simulink model "K_Sim_SG_Load"  (R2020b)
settings: Solver=FixedStepAuto  StartTime=0  StopTime=10  FixedStep=Ts  RelTol=1e-3
undefined symbols (not defined in the file or in its folder): DeviceDiscreDamping, DevicePara, DevicePowerFlow, DeviceType, Fbase, OtherInputs, Sbase, Ts, Vbase, Wbase, x_e, Ybase, Zbase
libraries: powerlib x222, SimplexPS x84
(part 1 of 2)
settings Model: Creator=admin_user  LastModifiedBy=admin_user

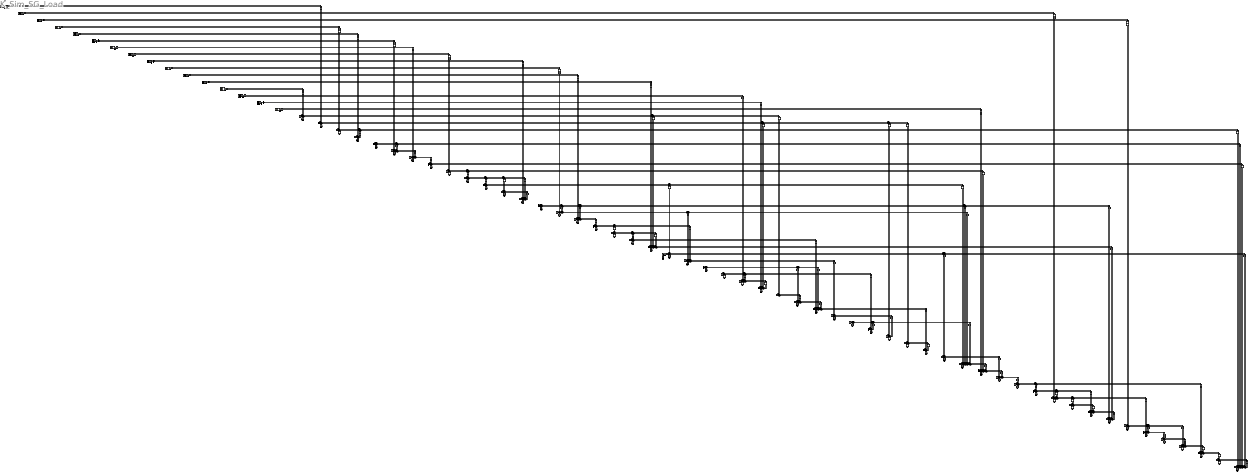
== system K_Sim_SG_Load ==
  note: Short-Circuit Fault
  B-GND{17,20,24,27..28,31,33,35,37,40,44,47,49..50,55,58,60,63,66,68,70,73,75,78,81,83,85,87,89,91,94..96,98..99,101,103,105,107,110,113,116,118,120..121,124,126,128,130,132,134} (51 alike) : powerlib/Elements/Ground  LConnTagsString=a
  Branch1-18 : powerlib/Elements/Three-Phase Series RLC Branch  LConnTagsString=A|B|C  RConnTagsString=A|B|C  BranchType=RL  Resistance=(1e-07)*Zbase  Inductance=(0.003)*Zbase/Wbase  Capacitance=1e-6  Measurements=None
  Branch10-31 : powerlib/Elements/Three-Phase Series RLC Branch  LConnTagsString=A|B|C  RConnTagsString=A|B|C  BranchType=RL  Resistance=(1e-07)*Zbase  Inductance=(0.026)*Zbase/Wbase  Capacitance=1e-6  Measurements=None
  Branch11-32 : powerlib/Elements/Three-Phase Series RLC Branch  LConnTagsString=A|B|C  RConnTagsString=A|B|C  BranchType=RL  Resistance=(1e-07)*Zbase  Inductance=(0.013)*Zbase/Wbase  Capacitance=1e-6  Measurements=None
  Branch12-36 : powerlib/Elements/Three-Phase Series RLC Branch  LConnTagsString=A|B|C  RConnTagsString=A|B|C  BranchType=RL  Resistance=(1e-07)*Zbase  Inductance=(0.0075)*Zbase/Wbase  Capacitance=1e-6  Measurements=None
  Branch13-17 : powerlib/Elements/Three-Phase Series RLC Branch  LConnTagsString=A|B|C  RConnTagsString=A|B|C  BranchType=RL  Resistance=(1e-07)*Zbase  Inductance=(0.0033)*Zbase/Wbase  Capacitance=1e-6  Measurements=None
  Branch14-41 : powerlib/Elements/Three-Phase Series RLC Branch  LConnTagsString=A|B|C  RConnTagsString=A|B|C  BranchType=RL  Resistance=(1e-07)*Zbase  Inductance=(0.0015)*Zbase/Wbase  Capacitance=1e-6  Measurements=None
  Branch15-42 : powerlib/Elements/Three-Phase Series RLC Branch  LConnTagsString=A|B|C  RConnTagsString=A|B|C  BranchType=RL  Resistance=(1e-07)*Zbase  Inductance=(0.0015)*Zbase/Wbase  Capacitance=1e-6  Measurements=None
  Branch16-54 : powerlib/Elements/Three-Phase Series RLC Branch  LConnTagsString=A|B|C  RConnTagsString=A|B|C  BranchType=RL  Resistance=(1e-07)*Zbase  Inductance=(0.0181)*Zbase/Wbase  Capacitance=1e-6  Measurements=None
  Branch17-17 : powerlib/Elements/Three-Phase Parallel RLC Branch  LConnTagsString=A|B|C  RConnTagsString=A|B|C  BranchType=RLC  Resistance=(0.015039)*Zbase  Inductance=(0.30078)*Zbase/Wbase  Capacitance=(0.16)*Ybase/Wbase  Measurements=None
      settings: SourceProductBaseCode=PS
  Branch17-36 : powerlib/Elements/Three-Phase Series RLC Branch  LConnTagsString=A|B|C  RConnTagsString=A|B|C  BranchType=RL  Resistance=(0.0005)*Zbase  Inductance=(0.0045)*Zbase/Wbase  Capacitance=1e-6  Measurements=None
  Branch17-43 : powerlib/Elements/Three-Phase Series RLC Branch  LConnTagsString=A|B|C  RConnTagsString=A|B|C  BranchType=RL  Resistance=(0.0005)*Zbase  Inductance=(0.0276)*Zbase/Wbase  Capacitance=1e-6  Measurements=None
  Branch18-18 : powerlib/Elements/Three-Phase Parallel RLC Branch  LConnTagsString=A|B|C  RConnTagsString=A|B|C  BranchType=RLC  Resistance=(0.040675)*Zbase  Inductance=(0.8168)*Zbase/Wbase  Capacitance=(2.735)*Ybase/Wbase  Measurements=None
      settings: SourceProductBaseCode=PS
  Branch18-42 : powerlib/Elements/Three-Phase Series RLC Branch  LConnTagsString=A|B|C  RConnTagsString=A|B|C  BranchType=RL  Resistance=(0.004)*Zbase  Inductance=(0.06)*Zbase/Wbase  Capacitance=1e-6  Measurements=None
  Branch18-49 : powerlib/Elements/Three-Phase Series RLC Branch  LConnTagsString=A|B|C  RConnTagsString=A|B|C  BranchType=RL  Resistance=(0.0076)*Zbase  Inductance=(0.1141)*Zbase/Wbase  Capacitance=1e-6  Measurements=None
  Branch18-50 : powerlib/Elements/Three-Phase Series RLC Branch  LConnTagsString=A|B|C  RConnTagsString=A|B|C  BranchType=RL  Resistance=(0.0012)*Zbase  Inductance=(0.0288)*Zbase/Wbase  Capacitance=1e-6  Measurements=None
  Branch19-19 : powerlib/Elements/Three-Phase Parallel RLC Branch  LConnTagsString=A|B|C  RConnTagsString=A|B|C  BranchType=C  Resistance=(Inf)*Zbase  Inductance=1e-3  Capacitance=(0.152)*Ybase/Wbase  Measurements=None
      settings: SourceProductBaseCode=PS
  Branch19-20 : powerlib/Elements/Three-Phase Series RLC Branch  LConnTagsString=A|B|C  RConnTagsString=A|B|C  BranchType=RL  Resistance=(0.00078652)*Zbase  Inductance=(0.015506)*Zbase/Wbase  Capacitance=1e-6  Measurements=None
  Branch19-68 : powerlib/Elements/Three-Phase Series RLC Branch  LConnTagsString=A|B|C  RConnTagsString=A|B|C  BranchType=RL  Resistance=(0.0016)*Zbase  Inductance=(0.0195)*Zbase/Wbase  Capacitance=1e-6  Measurements=None
  Branch2-58 : powerlib/Elements/Three-Phase Series RLC Branch  LConnTagsString=A|B|C  RConnTagsString=A|B|C  BranchType=RL  Resistance=(1e-07)*Zbase  Inductance=(0.025)*Zbase/Wbase  Capacitance=1e-6  Measurements=None
  Branch20-20 : powerlib/Elements/Three-Phase Parallel RLC Branch  LConnTagsString=A|B|C  RConnTagsString=A|B|C  BranchType=RL  Resistance=(0.14141)*Zbase  Inductance=(0.93359)*Zbase/Wbase  Capacitance=(0)*Ybase/Wbase  Measurements=None
      settings: SourceProductBaseCode=PS
  Branch21-21 : powerlib/Elements/Three-Phase Parallel RLC Branch  LConnTagsString=A|B|C  RConnTagsString=A|B|C  BranchType=RLC  Resistance=(0.33652)*Zbase  Inductance=(0.8018)*Zbase/Wbase  Capacitance=(0.25565)*Ybase/Wbase  Measurements=None
      settings: SourceProductBaseCode=PS
  Branch21-22 : powerlib/Elements/Three-Phase Series RLC Branch  LConnTagsString=A|B|C  RConnTagsString=A|B|C  BranchType=RL  Resistance=(0.0008)*Zbase  Inductance=(0.014)*Zbase/Wbase  Capacitance=1e-6  Measurements=None
  Branch21-68 : powerlib/Elements/Three-Phase Series RLC Branch  LConnTagsString=A|B|C  RConnTagsString=A|B|C  BranchType=RL  Resistance=(0.0008)*Zbase  Inductance=(0.0135)*Zbase/Wbase  Capacitance=1e-6  Measurements=None
  Branch22-22 : powerlib/Elements/Three-Phase Parallel RLC Branch  LConnTagsString=A|B|C  RConnTagsString=A|B|C  BranchType=C  Resistance=(Inf)*Zbase  Inductance=1e-3  Capacitance=(0.22055)*Ybase/Wbase  Measurements=None
      settings: SourceProductBaseCode=PS
  Branch22-23 : powerlib/Elements/Three-Phase Series RLC Branch  LConnTagsString=A|B|C  RConnTagsString=A|B|C  BranchType=RL  Resistance=(0.0006)*Zbase  Inductance=(0.0096)*Zbase/Wbase  Capacitance=1e-6  Measurements=None
  Branch23-23 : powerlib/Elements/Three-Phase Parallel RLC Branch  LConnTagsString=A|B|C  RConnTagsString=A|B|C  BranchType=RLC  Resistance=(0.40009)*Zbase  Inductance=(1.1673)*Zbase/Wbase  Capacitance=(0.2728)*Ybase/Wbase  Measurements=None
      settings: SourceProductBaseCode=PS
  Branch23-24 : powerlib/Elements/Three-Phase Series RLC Branch  LConnTagsString=A|B|C  RConnTagsString=A|B|C  BranchType=RL  Resistance=(0.0022)*Zbase  Inductance=(0.035)*Zbase/Wbase  Capacitance=1e-6  Measurements=None
  Branch24-24 : powerlib/Elements/Three-Phase Parallel RLC Branch  LConnTagsString=A|B|C  RConnTagsString=A|B|C  BranchType=RC  Resistance=(0.29745)*Zbase  Inductance=1e-3  Capacitance=(1.2155)*Ybase/Wbase  Measurements=None
      settings: SourceProductBaseCode=PS
  Branch24-68 : powerlib/Elements/Three-Phase Series RLC Branch  LConnTagsString=A|B|C  RConnTagsString=A|B|C  BranchType=RL  Resistance=(0.0003)*Zbase  Inductance=(0.0059)*Zbase/Wbase  Capacitance=1e-6  Measurements=None
  Branch25-25 : powerlib/Elements/Three-Phase Parallel RLC Branch  LConnTagsString=A|B|C  RConnTagsString=A|B|C  BranchType=RLC  Resistance=(0.44474)*Zbase  Inductance=(2.1196)*Zbase/Wbase  Capacitance=(0.3385)*Ybase/Wbase  Measurements=None
      settings: SourceProductBaseCode=PS
  Branch25-26 : powerlib/Elements/Three-Phase Series RLC Branch  LConnTagsString=A|B|C  RConnTagsString=A|B|C  BranchType=RL  Resistance=(0.0032)*Zbase  Inductance=(0.0323)*Zbase/Wbase  Capacitance=1e-6  Measurements=None
  Branch25-54 : powerlib/Elements/Three-Phase Series RLC Branch  LConnTagsString=A|B|C  RConnTagsString=A|B|C  BranchType=RL  Resistance=(0.007)*Zbase  Inductance=(0.0086)*Zbase/Wbase  Capacitance=1e-6  Measurements=None
  Branch26-26 : powerlib/Elements/Three-Phase Parallel RLC Branch  LConnTagsString=A|B|C  RConnTagsString=A|B|C  BranchType=RLC  Resistance=(0.70064)*Zbase  Inductance=(5.7288)*Zbase/Wbase  Capacitance=(1.2899)*Ybase/Wbase  Measurements=None
      settings: SourceProductBaseCode=PS
  Branch26-27 : powerlib/Elements/Three-Phase Series RLC Branch  LConnTagsString=A|B|C  RConnTagsString=A|B|C  BranchType=RL  Resistance=(0.0014)*Zbase  Inductance=(0.0147)*Zbase/Wbase  Capacitance=1e-6  Measurements=None
  Branch26-28 : powerlib/Elements/Three-Phase Series RLC Branch  LConnTagsString=A|B|C  RConnTagsString=A|B|C  BranchType=RL  Resistance=(0.0043)*Zbase  Inductance=(0.0474)*Zbase/Wbase  Capacitance=1e-6  Measurements=None
  Branch26-29 : powerlib/Elements/Three-Phase Series RLC Branch  LConnTagsString=A|B|C  RConnTagsString=A|B|C  BranchType=RL  Resistance=(0.0057)*Zbase  Inductance=(0.0625)*Zbase/Wbase  Capacitance=1e-6  Measurements=None
  Branch27-27 : powerlib/Elements/Three-Phase Parallel RLC Branch  LConnTagsString=A|B|C  RConnTagsString=A|B|C  BranchType=RLC  Resistance=(0.33339)*Zbase  Inductance=(1.2327)*Zbase/Wbase  Capacitance=(0.4856)*Ybase/Wbase  Measurements=None
      settings: SourceProductBaseCode=PS
  Branch27-37 : powerlib/Elements/Three-Phase Series RLC Branch  LConnTagsString=A|B|C  RConnTagsString=A|B|C  BranchType=RL  Resistance=(0.0013)*Zbase  Inductance=(0.0173)*Zbase/Wbase  Capacitance=1e-6  Measurements=None
  Branch27-53 : powerlib/Elements/Three-Phase Series RLC Branch  LConnTagsString=A|B|C  RConnTagsString=A|B|C  BranchType=RL  Resistance=(0.032)*Zbase  Inductance=(0.32)*Zbase/Wbase  Capacitance=1e-6  Measurements=None
  Branch28-28 : powerlib/Elements/Three-Phase Parallel RLC Branch  LConnTagsString=A|B|C  RConnTagsString=A|B|C  BranchType=RLC  Resistance=(0.47552)*Zbase  Inductance=(3.4985)*Zbase/Wbase  Capacitance=(0.5146)*Ybase/Wbase  Measurements=None
      settings: SourceProductBaseCode=PS
  Branch28-29 : powerlib/Elements/Three-Phase Series RLC Branch  LConnTagsString=A|B|C  RConnTagsString=A|B|C  BranchType=RL  Resistance=(0.0014)*Zbase  Inductance=(0.0151)*Zbase/Wbase  Capacitance=1e-6  Measurements=None
  Branch29-29 : powerlib/Elements/Three-Phase Parallel RLC Branch  LConnTagsString=A|B|C  RConnTagsString=A|B|C  BranchType=RLC  Resistance=(0.34656)*Zbase  Inductance=(3.6453)*Zbase/Wbase  Capacitance=(0.639)*Ybase/Wbase  Measurements=None
      settings: SourceProductBaseCode=PS
  Branch3-62 : powerlib/Elements/Three-Phase Series RLC Branch  LConnTagsString=A|B|C  RConnTagsString=A|B|C  BranchType=RL  Resistance=(1e-07)*Zbase  Inductance=(0.02)*Zbase/Wbase  Capacitance=1e-6  Measurements=None
  Branch30-30 : powerlib/Elements/Three-Phase Parallel RLC Branch  LConnTagsString=A|B|C  RConnTagsString=A|B|C  BranchType=C  Resistance=(Inf)*Zbase  Inductance=1e-3  Capacitance=(0.9405)*Ybase/Wbase  Measurements=None
      settings: SourceProductBaseCode=PS
  Branch30-31 : powerlib/Elements/Three-Phase Series RLC Branch  LConnTagsString=A|B|C  RConnTagsString=A|B|C  BranchType=RL  Resistance=(0.0013)*Zbase  Inductance=(0.0187)*Zbase/Wbase  Capacitance=1e-6  Measurements=None
  Branch30-32 : powerlib/Elements/Three-Phase Series RLC Branch  LConnTagsString=A|B|C  RConnTagsString=A|B|C  BranchType=RL  Resistance=(0.0024)*Zbase  Inductance=(0.0288)*Zbase/Wbase  Capacitance=1e-6  Measurements=None
  Branch30-53 : powerlib/Elements/Three-Phase Series RLC Branch  LConnTagsString=A|B|C  RConnTagsString=A|B|C  BranchType=RL  Resistance=(0.0008)*Zbase  Inductance=(0.0074)*Zbase/Wbase  Capacitance=1e-6  Measurements=None
  Branch30-61 : powerlib/Elements/Three-Phase Series RLC Branch  LConnTagsString=A|B|C  RConnTagsString=A|B|C  BranchType=RL  Resistance=(0.00095)*Zbase  Inductance=(0.00915)*Zbase/Wbase  Capacitance=1e-6  Measurements=None
  Branch31-31 : powerlib/Elements/Three-Phase Parallel RLC Branch  LConnTagsString=A|B|C  RConnTagsString=A|B|C  BranchType=C  Resistance=(Inf)*Zbase  Inductance=1e-3  Capacitance=(0.415)*Ybase/Wbase  Measurements=None
      settings: SourceProductBaseCode=PS
  Branch31-38 : powerlib/Elements/Three-Phase Series RLC Branch  LConnTagsString=A|B|C  RConnTagsString=A|B|C  BranchType=RL  Resistance=(0.0011)*Zbase  Inductance=(0.0147)*Zbase/Wbase  Capacitance=1e-6  Measurements=None
  Branch31-53 : powerlib/Elements/Three-Phase Series RLC Branch  LConnTagsString=A|B|C  RConnTagsString=A|B|C  BranchType=RL  Resistance=(0.0016)*Zbase  Inductance=(0.0163)*Zbase/Wbase  Capacitance=1e-6  Measurements=None
  Branch32-32 : powerlib/Elements/Three-Phase Parallel RLC Branch  LConnTagsString=A|B|C  RConnTagsString=A|B|C  BranchType=C  Resistance=(Inf)*Zbase  Inductance=1e-3  Capacitance=(0.328)*Ybase/Wbase  Measurements=None
      settings: SourceProductBaseCode=PS
  Branch32-33 : powerlib/Elements/Three-Phase Series RLC Branch  LConnTagsString=A|B|C  RConnTagsString=A|B|C  BranchType=RL  Resistance=(0.0008)*Zbase  Inductance=(0.0099)*Zbase/Wbase  Capacitance=1e-6  Measurements=None
  Branch33-33 : powerlib/Elements/Three-Phase Parallel RLC Branch  LConnTagsString=A|B|C  RConnTagsString=A|B|C  BranchType=RC  Resistance=(0.8467)*Zbase  Inductance=1e-3  Capacitance=(0.5315)*Ybase/Wbase  Measurements=None
      settings: SourceProductBaseCode=PS
  Branch33-34 : powerlib/Elements/Three-Phase Series RLC Branch  LConnTagsString=A|B|C  RConnTagsString=A|B|C  BranchType=RL  Resistance=(0.0011)*Zbase  Inductance=(0.0157)*Zbase/Wbase  Capacitance=1e-6  Measurements=None
  Branch33-38 : powerlib/Elements/Three-Phase Series RLC Branch  LConnTagsString=A|B|C  RConnTagsString=A|B|C  BranchType=RL  Resistance=(0.0036)*Zbase  Inductance=(0.0444)*Zbase/Wbase  Capacitance=1e-6  Measurements=None
  Branch34-34 : powerlib/Elements/Three-Phase Parallel RLC Branch  LConnTagsString=A|B|C  RConnTagsString=A|B|C  BranchType=C  Resistance=(Inf)*Zbase  Inductance=1e-3  Capacitance=(0.826)*Ybase/Wbase  Measurements=None
      settings: SourceProductBaseCode=PS
  Branch34-35 : powerlib/Elements/Three-Phase Series RLC Branch  LConnTagsString=A|B|C  RConnTagsString=A|B|C  BranchType=RL  Resistance=(0.0001)*Zbase  Inductance=(0.0074)*Zbase/Wbase  Capacitance=1e-6  Measurements=None
  Branch34-36 : powerlib/Elements/Three-Phase Series RLC Branch  LConnTagsString=A|B|C  RConnTagsString=A|B|C  BranchType=RL  Resistance=(0.0033)*Zbase  Inductance=(0.0111)*Zbase/Wbase  Capacitance=1e-6  Measurements=None
  Branch35-35 : powerlib/Elements/Three-Phase Parallel RLC Branch  LConnTagsString=A|B|C  RConnTagsString=A|B|C  BranchType=C  Resistance=(Inf)*Zbase  Inductance=1e-3  Capacitance=(0.695)*Ybase/Wbase  Measurements=None
      settings: SourceProductBaseCode=PS
  Branch35-45 : powerlib/Elements/Three-Phase Series RLC Branch  LConnTagsString=A|B|C  RConnTagsString=A|B|C  BranchType=RL  Resistance=(0.0007)*Zbase  Inductance=(0.0175)*Zbase/Wbase  Capacitance=1e-6  Measurements=None
  Branch36-36 : powerlib/Elements/Three-Phase Parallel RLC Branch  LConnTagsString=A|B|C  RConnTagsString=A|B|C  BranchType=RC  Resistance=(0.90473)*Zbase  Inductance=1e-3  Capacitance=(1.4359)*Ybase/Wbase  Measurements=None
      settings: SourceProductBaseCode=PS
  Branch36-61 : powerlib/Elements/Three-Phase Series RLC Branch  LConnTagsString=A|B|C  RConnTagsString=A|B|C  BranchType=RL  Resistance=(0.0011)*Zbase  Inductance=(0.0098)*Zbase/Wbase  Capacitance=1e-6  Measurements=None
  Branch37-37 : powerlib/Elements/Three-Phase Parallel RLC Branch  LConnTagsString=A|B|C  RConnTagsString=A|B|C  BranchType=C  Resistance=(Inf)*Zbase  Inductance=1e-3  Capacitance=(0.29385)*Ybase/Wbase  Measurements=None
      settings: SourceProductBaseCode=PS
  Branch37-52 : powerlib/Elements/Three-Phase Series RLC Branch  LConnTagsString=A|B|C  RConnTagsString=A|B|C  BranchType=RL  Resistance=(0.0007)*Zbase  Inductance=(0.0082)*Zbase/Wbase  Capacitance=1e-6  Measurements=None
  Branch37-68 : powerlib/Elements/Three-Phase Series RLC Branch  LConnTagsString=A|B|C  RConnTagsString=A|B|C  BranchType=RL  Resistance=(0.0007)*Zbase  Inductance=(0.0089)*Zbase/Wbase  Capacitance=1e-6  Measurements=None
  Branch38-38 : powerlib/Elements/Three-Phase Parallel RLC Branch  LConnTagsString=A|B|C  RConnTagsString=A|B|C  BranchType=C  Resistance=(Inf)*Zbase  Inductance=1e-3  Capacitance=(0.685)*Ybase/Wbase  Measurements=None
      settings: SourceProductBaseCode=PS
  Branch38-46 : powerlib/Elements/Three-Phase Series RLC Branch  LConnTagsString=A|B|C  RConnTagsString=A|B|C  BranchType=RL  Resistance=(0.0022)*Zbase  Inductance=(0.0284)*Zbase/Wbase  Capacitance=1e-6  Measurements=None
  Branch39-39 : powerlib/Elements/Three-Phase Parallel RLC Branch  LConnTagsString=A|B|C  RConnTagsString=A|B|C  BranchType=RL  Resistance=(0.36822)*Zbase  Inductance=(7.8028)*Zbase/Wbase  Capacitance=(0)*Ybase/Wbase  Measurements=None
      settings: SourceProductBaseCode=PS
  Branch39-44 : powerlib/Elements/Three-Phase Series RLC Branch  LConnTagsString=A|B|C  RConnTagsString=A|B|C  BranchType=RL  Resistance=(1e-07)*Zbase  Inductance=(0.0411)*Zbase/Wbase  Capacitance=1e-6  Measurements=None
  Branch39-45 : powerlib/Elements/Three-Phase Series RLC Branch  LConnTagsString=A|B|C  RConnTagsString=A|B|C  BranchType=RL  Resistance=(1e-07)*Zbase  Inductance=(0.0839)*Zbase/Wbase  Capacitance=1e-6  Measurements=None
  Branch4-19 : powerlib/Elements/Three-Phase Series RLC Branch  LConnTagsString=A|B|C  RConnTagsString=A|B|C  BranchType=RL  Resistance=(0.0007)*Zbase  Inductance=(0.0142)*Zbase/Wbase  Capacitance=1e-6  Measurements=None
  Branch40-40 : powerlib/Elements/Three-Phase Parallel RLC Branch  LConnTagsString=A|B|C  RConnTagsString=A|B|C  BranchType=RLC  Resistance=(1.6614)*Zbase  Inductance=(4.6341)*Zbase/Wbase  Capacitance=(2.215)*Ybase/Wbase  Measurements=None
      settings: SourceProductBaseCode=PS
  Branch40-41 : powerlib/Elements/Three-Phase Series RLC Branch  LConnTagsString=A|B|C  RConnTagsString=A|B|C  BranchType=RL  Resistance=(0.006)*Zbase  Inductance=(0.084)*Zbase/Wbase  Capacitance=1e-6  Measurements=None
  Branch40-48 : powerlib/Elements/Three-Phase Series RLC Branch  LConnTagsString=A|B|C  RConnTagsString=A|B|C  BranchType=RL  Resistance=(0.002)*Zbase  Inductance=(0.022)*Zbase/Wbase  Capacitance=1e-6  Measurements=None
  Branch41-41 : powerlib/Elements/Three-Phase Parallel RLC Branch  LConnTagsString=A|B|C  RConnTagsString=A|B|C  BranchType=RLC  Resistance=(0.099929)*Zbase  Inductance=(0.39972)*Zbase/Wbase  Capacitance=(2.7)*Ybase/Wbase  Measurements=None
      settings: SourceProductBaseCode=PS
  Branch41-42 : powerlib/Elements/Three-Phase Series RLC Branch  LConnTagsString=A|B|C  RConnTagsString=A|B|C  BranchType=RL  Resistance=(0.004)*Zbase  Inductance=(0.06)*Zbase/Wbase  Capacitance=1e-6  Measurements=None
  Branch42-42 : powerlib/Elements/Three-Phase Parallel RLC Branch  LConnTagsString=A|B|C  RConnTagsString=A|B|C  BranchType=RLC  Resistance=(0.086776)*Zbase  Inductance=(0.39917)*Zbase/Wbase  Capacitance=(2.25)*Ybase/Wbase  Measurements=None
      settings: SourceProductBaseCode=PS
  Branch43-44 : powerlib/Elements/Three-Phase Series RLC Branch  LConnTagsString=A|B|C  RConnTagsString=A|B|C  BranchType=RL  Resistance=(0.0001)*Zbase  Inductance=(0.0011)*Zbase/Wbase  Capacitance=1e-6  Measurements=None
  Branch44-44 : powerlib/Elements/Three-Phase Parallel RLC Branch  LConnTagsString=A|B|C  RConnTagsString=A|B|C  BranchType=RL  Resistance=(0.35712)*Zbase  Inductance=(19.7413)*Zbase/Wbase  Capacitance=(0)*Ybase/Wbase  Measurements=None
      settings: SourceProductBaseCode=PS
  Branch44-45 : powerlib/Elements/Three-Phase Series RLC Branch  LConnTagsString=A|B|C  RConnTagsString=A|B|C  BranchType=RL  Resistance=(0.0025)*Zbase  Inductance=(0.073)*Zbase/Wbase  Capacitance=1e-6  Measurements=None
  Branch45-45 : powerlib/Elements/Three-Phase Parallel RLC Branch  LConnTagsString=A|B|C  RConnTagsString=A|B|C  BranchType=RLC  Resistance=(0.52711)*Zbase  Inductance=(5.2209)*Zbase/Wbase  Capacitance=(1.055)*Ybase/Wbase  Measurements=None
      settings: SourceProductBaseCode=PS
  Branch45-51 : powerlib/Elements/Three-Phase Series RLC Branch  LConnTagsString=A|B|C  RConnTagsString=A|B|C  BranchType=RL  Resistance=(0.0004)*Zbase  Inductance=(0.0105)*Zbase/Wbase  Capacitance=1e-6  Measurements=None
  Branch46-46 : powerlib/Elements/Three-Phase Parallel RLC Branch  LConnTagsString=A|B|C  RConnTagsString=A|B|C  BranchType=RLC  Resistance=(0.65078)*Zbase  Inductance=(3.4411)*Zbase/Wbase  Capacitance=(0.35)*Ybase/Wbase  Measurements=None
      settings: SourceProductBaseCode=PS
  Branch46-49 : powerlib/Elements/Three-Phase Series RLC Branch  LConnTagsString=A|B|C  RConnTagsString=A|B|C  BranchType=RL  Resistance=(0.0018)*Zbase  Inductance=(0.0274)*Zbase/Wbase  Capacitance=1e-6  Measurements=None
  Branch47-47 : powerlib/Elements/Three-Phase Parallel RLC Branch  LConnTagsString=A|B|C  RConnTagsString=A|B|C  BranchType=RLC  Resistance=(0.5106)*Zbase  Inductance=(3.1824)*Zbase/Wbase  Capacitance=(1.055)*Ybase/Wbase  Measurements=None
      settings: SourceProductBaseCode=PS
  Branch47-48 : powerlib/Elements/Three-Phase Series RLC Branch  LConnTagsString=A|B|C  RConnTagsString=A|B|C  BranchType=RL  Resistance=(0.00125)*Zbase  Inductance=(0.0134)*Zbase/Wbase  Capacitance=1e-6  Measurements=None
  Branch47-53 : powerlib/Elements/Three-Phase Series RLC Branch  LConnTagsString=A|B|C  RConnTagsString=A|B|C  BranchType=RL  Resistance=(0.0013)*Zbase  Inductance=(0.0188)*Zbase/Wbase  Capacitance=1e-6  Measurements=None
  Branch48-48 : powerlib/Elements/Three-Phase Parallel RLC Branch  LConnTagsString=A|B|C  RConnTagsString=A|B|C  BranchType=RLC  Resistance=(0.44304)*Zbase  Inductance=(48.5738)*Zbase/Wbase  Capacitance=(1.04)*Ybase/Wbase  Measurements=None
      settings: SourceProductBaseCode=PS
  Branch49-49 : powerlib/Elements/Three-Phase Parallel RLC Branch  LConnTagsString=A|B|C  RConnTagsString=A|B|C  BranchType=RLC  Resistance=(0.60199)*Zbase  Inductance=(3.4044)*Zbase/Wbase  Capacitance=(0.715)*Ybase/Wbase  Measurements=None
      settings: SourceProductBaseCode=PS
  Branch5-20 : powerlib/Elements/Three-Phase Series RLC Branch  LConnTagsString=A|B|C  RConnTagsString=A|B|C  BranchType=RL  Resistance=(0.0009)*Zbase  Inductance=(0.018)*Zbase/Wbase  Capacitance=1e-6  Measurements=None
  Branch50-50 : powerlib/Elements/Three-Phase Parallel RLC Branch  LConnTagsString=A|B|C  RConnTagsString=A|B|C  BranchType=RC  Resistance=(1.1241)*Zbase  Inductance=1e-3  Capacitance=(3.1477)*Ybase/Wbase  Measurements=None
      settings: SourceProductBaseCode=PS
  Branch50-51 : powerlib/Elements/Three-Phase Series RLC Branch  LConnTagsString=A|B|C  RConnTagsString=A|B|C  BranchType=RL  Resistance=(0.0009)*Zbase  Inductance=(0.0221)*Zbase/Wbase  Capacitance=1e-6  Measurements=None
  Branch51-51 : powerlib/Elements/Three-Phase Parallel RLC Branch  LConnTagsString=A|B|C  RConnTagsString=A|B|C  BranchType=RC  Resistance=(0.33554)*Zbase  Inductance=1e-3  Capacitance=(2.2489)*Ybase/Wbase  Measurements=None
      settings: SourceProductBaseCode=PS
  Branch52-52 : powerlib/Elements/Three-Phase Parallel RLC Branch  LConnTagsString=A|B|C  RConnTagsString=A|B|C  BranchType=RLC  Resistance=(0.57667)*Zbase  Inductance=(3.0371)*Zbase/Wbase  Capacitance=(0.17285)*Ybase/Wbase  Measurements=None
      settings: SourceProductBaseCode=PS
  Branch52-55 : powerlib/Elements/Three-Phase Series RLC Branch  LConnTagsString=A|B|C  RConnTagsString=A|B|C  BranchType=RL  Resistance=(0.0011)*Zbase  Inductance=(0.0133)*Zbase/Wbase  Capacitance=1e-6  Measurements=None
  Branch53-53 : powerlib/Elements/Three-Phase Parallel RLC Branch  LConnTagsString=A|B|C  RConnTagsString=A|B|C  BranchType=RLC  Resistance=(0.38498)*Zbase  Inductance=(0.82056)*Zbase/Wbase  Capacitance=(1.5744)*Ybase/Wbase  Measurements=None
      settings: SourceProductBaseCode=PS
  Branch53-54 : powerlib/Elements/Three-Phase Series RLC Branch  LConnTagsString=A|B|C  RConnTagsString=A|B|C  BranchType=RL  Resistance=(0.0035)*Zbase  Inductance=(0.0411)*Zbase/Wbase  Capacitance=1e-6  Measurements=None
  Branch54-54 : powerlib/Elements/Three-Phase Parallel RLC Branch  LConnTagsString=A|B|C  RConnTagsString=A|B|C  BranchType=C  Resistance=(Inf)*Zbase  Inductance=1e-3  Capacitance=(0.55095)*Ybase/Wbase  Measurements=None
      settings: SourceProductBaseCode=PS
  Branch54-55 : powerlib/Elements/Three-Phase Series RLC Branch  LConnTagsString=A|B|C  RConnTagsString=A|B|C  BranchType=RL  Resistance=(0.0013)*Zbase  Inductance=(0.0151)*Zbase/Wbase  Capacitance=1e-6  Measurements=None
  Branch55-55 : powerlib/Elements/Three-Phase Parallel RLC Branch  LConnTagsString=A|B|C  RConnTagsString=A|B|C  BranchType=RLC  Resistance=(0.2845)*Zbase  Inductance=(45.8038)*Zbase/Wbase  Capacitance=(0.3462)*Ybase/Wbase  Measurements=None
      settings: SourceProductBaseCode=PS
  Branch55-56 : powerlib/Elements/Three-Phase Series RLC Branch  LConnTagsString=A|B|C  RConnTagsString=A|B|C  BranchType=RL  Resistance=(0.0013)*Zbase  Inductance=(0.0213)*Zbase/Wbase  Capacitance=1e-6  Measurements=None
  Branch56-56 : powerlib/Elements/Three-Phase Parallel RLC Branch  LConnTagsString=A|B|C  RConnTagsString=A|B|C  BranchType=RLC  Resistance=(0.42398)*Zbase  Inductance=(1.1521)*Zbase/Wbase  Capacitance=(0.2469)*Ybase/Wbase  Measurements=None
      settings: SourceProductBaseCode=PS
  Branch56-57 : powerlib/Elements/Three-Phase Series RLC Branch  LConnTagsString=A|B|C  RConnTagsString=A|B|C  BranchType=RL  Resistance=(0.0008)*Zbase  Inductance=(0.0128)*Zbase/Wbase  Capacitance=1e-6  Measurements=None
  Branch56-66 : powerlib/Elements/Three-Phase Series RLC Branch  LConnTagsString=A|B|C  RConnTagsString=A|B|C  BranchType=RL  Resistance=(0.0008)*Zbase  Inductance=(0.0129)*Zbase/Wbase  Capacitance=1e-6  Measurements=None
  Branch57-57 : powerlib/Elements/Three-Phase Parallel RLC Branch  LConnTagsString=A|B|C  RConnTagsString=A|B|C  BranchType=C  Resistance=(Inf)*Zbase  Inductance=1e-3  Capacitance=(0.1626)*Ybase/Wbase  Measurements=None
      settings: SourceProductBaseCode=PS
  Branch57-58 : powerlib/Elements/Three-Phase Series RLC Branch  LConnTagsString=A|B|C  RConnTagsString=A|B|C  BranchType=RL  Resistance=(0.0002)*Zbase  Inductance=(0.0026)*Zbase/Wbase  Capacitance=1e-6  Measurements=None
  Branch57-60 : powerlib/Elements/Three-Phase Series RLC Branch  LConnTagsString=A|B|C  RConnTagsString=A|B|C  BranchType=RL  Resistance=(0.0008)*Zbase  Inductance=(0.0112)*Zbase/Wbase  Capacitance=1e-6  Measurements=None
  Branch58-58 : powerlib/Elements/Three-Phase Parallel RLC Branch  LConnTagsString=A|B|C  RConnTagsString=A|B|C  BranchType=C  Resistance=(Inf)*Zbase  Inductance=1e-3  Capacitance=(0.14765)*Ybase/Wbase  Measurements=None
      settings: SourceProductBaseCode=PS
  Branch58-59 : powerlib/Elements/Three-Phase Series RLC Branch  LConnTagsString=A|B|C  RConnTagsString=A|B|C  BranchType=RL  Resistance=(0.0006)*Zbase  Inductance=(0.0092)*Zbase/Wbase  Capacitance=1e-6  Measurements=None
  Branch58-63 : powerlib/Elements/Three-Phase Series RLC Branch  LConnTagsString=A|B|C  RConnTagsString=A|B|C  BranchType=RL  Resistance=(0.0007)*Zbase  Inductance=(0.0082)*Zbase/Wbase  Capacitance=1e-6  Measurements=None
  Branch59-59 : powerlib/Elements/Three-Phase Parallel RLC Branch  LConnTagsString=A|B|C  RConnTagsString=A|B|C  BranchType=RLC  Resistance=(0.34904)*Zbase  Inductance=(0.97233)*Zbase/Wbase  Capacitance=(0.0955)*Ybase/Wbase  Measurements=None
      settings: SourceProductBaseCode=PS
  Branch59-60 : powerlib/Elements/Three-Phase Series RLC Branch  LConnTagsString=A|B|C  RConnTagsString=A|B|C  BranchType=RL  Resistance=(0.0004)*Zbase  Inductance=(0.0046)*Zbase/Wbase  Capacitance=1e-6  Measurements=None
  Branch6-22 : powerlib/Elements/Three-Phase Series RLC Branch  LConnTagsString=A|B|C  RConnTagsString=A|B|C  BranchType=RL  Resistance=(1e-07)*Zbase  Inductance=(0.0143)*Zbase/Wbase  Capacitance=1e-6  Measurements=None
  Branch60-60 : powerlib/Elements/Three-Phase Parallel RLC Branch  LConnTagsString=A|B|C  RConnTagsString=A|B|C  BranchType=RLC  Resistance=(0.39327)*Zbase  Inductance=(1.1598)*Zbase/Wbase  Capacitance=(0.303)*Ybase/Wbase  Measurements=None
      settings: SourceProductBaseCode=PS
  Branch60-61 : powerlib/Elements/Three-Phase Series RLC Branch  LConnTagsString=A|B|C  RConnTagsString=A|B|C  BranchType=RL  Resistance=(0.0023)*Zbase  Inductance=(0.0363)*Zbase/Wbase  Capacitance=1e-6  Measurements=None
  Branch61-61 : powerlib/Elements/Three-Phase Parallel RLC Branch  LConnTagsString=A|B|C  RConnTagsString=A|B|C  BranchType=RLC  Resistance=(0.87814)*Zbase  Inductance=(0.73061)*Zbase/Wbase  Capacitance=(0.8202)*Ybase/Wbase  Measurements=None
      settings: SourceProductBaseCode=PS
  Branch62-62 : powerlib/Elements/Three-Phase Parallel RLC Branch  LConnTagsString=A|B|C  RConnTagsString=A|B|C  BranchType=C  Resistance=(Inf)*Zbase  Inductance=1e-3  Capacitance=(0.0729)*Ybase/Wbase  Measurements=None
      settings: SourceProductBaseCode=PS
  Branch62-63 : powerlib/Elements/Three-Phase Series RLC Branch  LConnTagsString=A|B|C  RConnTagsString=A|B|C  BranchType=RL  Resistance=(0.0004)*Zbase  Inductance=(0.0043)*Zbase/Wbase  Capacitance=1e-6  Measurements=None
  Branch62-65 : powerlib/Elements/Three-Phase Series RLC Branch  LConnTagsString=A|B|C  RConnTagsString=A|B|C  BranchType=RL  Resistance=(0.0004)*Zbase  Inductance=(0.0043)*Zbase/Wbase  Capacitance=1e-6  Measurements=None
  Branch63-63 : powerlib/Elements/Three-Phase Parallel RLC Branch  LConnTagsString=A|B|C  RConnTagsString=A|B|C  BranchType=C  Resistance=(Inf)*Zbase  Inductance=1e-3  Capacitance=(0.1059)*Ybase/Wbase  Measurements=None
      settings: SourceProductBaseCode=PS
  Branch63-64 : powerlib/Elements/Three-Phase Series RLC Branch  LConnTagsString=A|B|C  RConnTagsString=A|B|C  BranchType=RL  Resistance=(0.0016)*Zbase  Inductance=(0.0435)*Zbase/Wbase  Capacitance=1e-6  Measurements=None
  Branch64-64 : powerlib/Elements/Three-Phase Parallel RLC Branch  LConnTagsString=A|B|C  RConnTagsString=A|B|C  BranchType=RL  Resistance=(7.7778)*Zbase  Inductance=(0.79545)*Zbase/Wbase  Capacitance=(0)*Ybase/Wbase  Measurements=None
      settings: SourceProductBaseCode=PS
  Branch64-65 : powerlib/Elements/Three-Phase Series RLC Branch  LConnTagsString=A|B|C  RConnTagsString=A|B|C  BranchType=RL  Resistance=(0.0017978)*Zbase  Inductance=(0.048877)*Zbase/Wbase  Capacitance=1e-6  Measurements=None
  Branch65-65 : powerlib/Elements/Three-Phase Parallel RLC Branch  LConnTagsString=A|B|C  RConnTagsString=A|B|C  BranchType=C  Resistance=(Inf)*Zbase  Inductance=1e-3  Capacitance=(0.1226)*Ybase/Wbase  Measurements=None
      settings: SourceProductBaseCode=PS
  Branch65-66 : powerlib/Elements/Three-Phase Series RLC Branch  LConnTagsString=A|B|C  RConnTagsString=A|B|C  BranchType=RL  Resistance=(0.0009)*Zbase  Inductance=(0.0101)*Zbase/Wbase  Capacitance=1e-6  Measurements=None
  Branch66-66 : powerlib/Elements/Three-Phase Parallel RLC Branch  LConnTagsString=A|B|C  RConnTagsString=A|B|C  BranchType=C  Resistance=(Inf)*Zbase  Inductance=1e-3  Capacitance=(0.33825)*Ybase/Wbase  Measurements=None
      settings: SourceProductBaseCode=PS
  Branch66-67 : powerlib/Elements/Three-Phase Series RLC Branch  LConnTagsString=A|B|C  RConnTagsString=A|B|C  BranchType=RL  Resistance=(0.0018)*Zbase  Inductance=(0.0217)*Zbase/Wbase  Capacitance=1e-6  Measurements=None
  Branch67-67 : powerlib/Elements/Three-Phase Parallel RLC Branch  LConnTagsString=A|B|C  RConnTagsString=A|B|C  BranchType=RLC  Resistance=(0.26914)*Zbase  Inductance=(0.56291)*Zbase/Wbase  Capacitance=(0.2685)*Ybase/Wbase  Measurements=None
      settings: SourceProductBaseCode=PS
  Branch67-68 : powerlib/Elements/Three-Phase Series RLC Branch  LConnTagsString=A|B|C  RConnTagsString=A|B|C  BranchType=RL  Resistance=(0.0009)*Zbase  Inductance=(0.0094)*Zbase/Wbase  Capacitance=1e-6  Measurements=None
  Branch68-68 : powerlib/Elements/Three-Phase Parallel RLC Branch  LConnTagsString=A|B|C  RConnTagsString=A|B|C  BranchType=RLC  Resistance=(0.27333)*Zbase  Inductance=(2.8102)*Zbase/Wbase  Capacitance=(0.466)*Ybase/Wbase  Measurements=None
      settings: SourceProductBaseCode=PS
  Branch7-23 : powerlib/Elements/Three-Phase Series RLC Branch  LConnTagsString=A|B|C  RConnTagsString=A|B|C  BranchType=RL  Resistance=(0.0005)*Zbase  Inductance=(0.0272)*Zbase/Wbase  Capacitance=1e-6  Measurements=None
  Branch8-25 : powerlib/Elements/Three-Phase Series RLC Branch  LConnTagsString=A|B|C  RConnTagsString=A|B|C  BranchType=RL  Resistance=(0.0006)*Zbase  Inductance=(0.0232)*Zbase/Wbase  Capacitance=1e-6  Measurements=None
  Branch9-29 : powerlib/Elements/Three-Phase Series RLC Branch  LConnTagsString=A|B|C  RConnTagsString=A|B|C  BranchType=RL  Resistance=(0.0008)*Zbase  Inductance=(0.0156)*Zbase/Wbase  Capacitance=1e-6  Measurements=None
  Bus{1..68} (68 alike) : SimplexPS/Three-Phase Bus  Vbase=1  Sbase=1
  Current Measurement1 : powerlib/Measurements/Current Measurement  PhasorSimulation=off  OutputType=Complex  PSBequivalent=0
  D-GND{1..16,22} (17 alike) : powerlib/Elements/Ground  LConnTagsString=a
  D-Scope{1..16} (16 alike) : Scope  NumInputPorts=7
  DS-Bus{1..16} (16 alike) : BusSelector  OutputSignals=v_dq,i_dq,v_abc,i_abc,w,theta,pq
  Load Impulse1 : Subsystem  AncestorBlock=SimplexPS/Load Impulse  mask{t0=2.5, dt=3/60, R=1e-9*Zbase}
  SM1 : SimplexPS/Synchronous Machine (dq-Frame System Object)  Ts=Ts  Sbase=Sbase  Vbase=Vbase  Wbase=Wbase  DeviceType=DeviceType{1}  DevicePara=DevicePara{1}  PowerFlow=DevicePowerFlow{1}  x0=x_e{1}  OtherInputs=OtherInputs{1}  DiscreMethod=Hybrid Trapezoidal  EnableInsideModification=off  DiscreDampingFlag=on  DiscreDampingValue=DeviceDiscreDamping{1}  LinearizationTimes=1  DirectFeedthrough=off
  SM10 : SimplexPS/Synchronous Machine (dq-Frame System Object)  Ts=Ts  Sbase=Sbase  Vbase=Vbase  Wbase=Wbase  DeviceType=DeviceType{10}  DevicePara=DevicePara{10}  PowerFlow=DevicePowerFlow{10}  x0=x_e{10}  OtherInputs=OtherInputs{10}  DiscreMethod=Hybrid Trapezoidal  EnableInsideModification=off  DiscreDampingFlag=on  DiscreDampingValue=DeviceDiscreDamping{10}  LinearizationTimes=1  DirectFeedthrough=off
  SM11 : SimplexPS/Synchronous Machine (dq-Frame System Object)  Ts=Ts  Sbase=Sbase  Vbase=Vbase  Wbase=Wbase  DeviceType=DeviceType{11}  DevicePara=DevicePara{11}  PowerFlow=DevicePowerFlow{11}  x0=x_e{11}  OtherInputs=OtherInputs{11}  DiscreMethod=Hybrid Trapezoidal  EnableInsideModification=off  DiscreDampingFlag=on  DiscreDampingValue=DeviceDiscreDamping{11}  LinearizationTimes=1  DirectFeedthrough=off
  SM12 : SimplexPS/Synchronous Machine (dq-Frame System Object)  Ts=Ts  Sbase=Sbase  Vbase=Vbase  Wbase=Wbase  DeviceType=DeviceType{12}  DevicePara=DevicePara{12}  PowerFlow=DevicePowerFlow{12}  x0=x_e{12}  OtherInputs=OtherInputs{12}  DiscreMethod=Hybrid Trapezoidal  EnableInsideModification=off  DiscreDampingFlag=on  DiscreDampingValue=DeviceDiscreDamping{12}  LinearizationTimes=1  DirectFeedthrough=off
  SM13 : SimplexPS/Synchronous Machine (dq-Frame System Object)  Ts=Ts  Sbase=Sbase  Vbase=Vbase  Wbase=Wbase  DeviceType=DeviceType{13}  DevicePara=DevicePara{13}  PowerFlow=DevicePowerFlow{13}  x0=x_e{13}  OtherInputs=OtherInputs{13}  DiscreMethod=Hybrid Trapezoidal  EnableInsideModification=off  DiscreDampingFlag=on  DiscreDampingValue=DeviceDiscreDamping{13}  LinearizationTimes=1  DirectFeedthrough=off
  SM14 : SimplexPS/Synchronous Machine (dq-Frame System Object)  Ts=Ts  Sbase=Sbase  Vbase=Vbase  Wbase=Wbase  DeviceType=DeviceType{14}  DevicePara=DevicePara{14}  PowerFlow=DevicePowerFlow{14}  x0=x_e{14}  OtherInputs=OtherInputs{14}  DiscreMethod=Hybrid Trapezoidal  EnableInsideModification=off  DiscreDampingFlag=on  DiscreDampingValue=DeviceDiscreDamping{14}  LinearizationTimes=1  DirectFeedthrough=off
  SM15 : SimplexPS/Synchronous Machine (dq-Frame System Object)  Ts=Ts  Sbase=Sbase  Vbase=Vbase  Wbase=Wbase  DeviceType=DeviceType{15}  DevicePara=DevicePara{15}  PowerFlow=DevicePowerFlow{15}  x0=x_e{15}  OtherInputs=OtherInputs{15}  DiscreMethod=Hybrid Trapezoidal  EnableInsideModification=off  DiscreDampingFlag=on  DiscreDampingValue=DeviceDiscreDamping{15}  LinearizationTimes=1  DirectFeedthrough=off
  SM16 : SimplexPS/Synchronous Machine (dq-Frame System Object)  Ts=Ts  Sbase=Sbase  Vbase=Vbase  Wbase=Wbase  DeviceType=DeviceType{16}  DevicePara=DevicePara{16}  PowerFlow=DevicePowerFlow{16}  x0=x_e{16}  OtherInputs=OtherInputs{16}  DiscreMethod=Hybrid Trapezoidal  EnableInsideModification=off  DiscreDampingFlag=on  DiscreDampingValue=DeviceDiscreDamping{16}  LinearizationTimes=1  DirectFeedthrough=off
  SM2 : SimplexPS/Synchronous Machine (dq-Frame System Object)  Ts=Ts  Sbase=Sbase  Vbase=Vbase  Wbase=Wbase  DeviceType=DeviceType{2}  DevicePara=DevicePara{2}  PowerFlow=DevicePowerFlow{2}  x0=x_e{2}  OtherInputs=OtherInputs{2}  DiscreMethod=Hybrid Trapezoidal  EnableInsideModification=off  DiscreDampingFlag=on  DiscreDampingValue=DeviceDiscreDamping{2}  LinearizationTimes=1  DirectFeedthrough=off
  SM3 : SimplexPS/Synchronous Machine (dq-Frame System Object)  Ts=Ts  Sbase=Sbase  Vbase=Vbase  Wbase=Wbase  DeviceType=DeviceType{3}  DevicePara=DevicePara{3}  PowerFlow=DevicePowerFlow{3}  x0=x_e{3}  OtherInputs=OtherInputs{3}  DiscreMethod=Hybrid Trapezoidal  EnableInsideModification=off  DiscreDampingFlag=on  DiscreDampingValue=DeviceDiscreDamping{3}  LinearizationTimes=1  DirectFeedthrough=off
  SM4 : SimplexPS/Synchronous Machine (dq-Frame System Object)  Ts=Ts  Sbase=Sbase  Vbase=Vbase  Wbase=Wbase  DeviceType=DeviceType{4}  DevicePara=DevicePara{4}  PowerFlow=DevicePowerFlow{4}  x0=x_e{4}  OtherInputs=OtherInputs{4}  DiscreMethod=Hybrid Trapezoidal  EnableInsideModification=off  DiscreDampingFlag=on  DiscreDampingValue=DeviceDiscreDamping{4}  LinearizationTimes=1  DirectFeedthrough=off
  SM5 : SimplexPS/Synchronous Machine (dq-Frame System Object)  Ts=Ts  Sbase=Sbase  Vbase=Vbase  Wbase=Wbase  DeviceType=DeviceType{5}  DevicePara=DevicePara{5}  PowerFlow=DevicePowerFlow{5}  x0=x_e{5}  OtherInputs=OtherInputs{5}  DiscreMethod=Hybrid Trapezoidal  EnableInsideModification=off  DiscreDampingFlag=on  DiscreDampingValue=DeviceDiscreDamping{5}  LinearizationTimes=1  DirectFeedthrough=off
  SM6 : SimplexPS/Synchronous Machine (dq-Frame System Object)  Ts=Ts  Sbase=Sbase  Vbase=Vbase  Wbase=Wbase  DeviceType=DeviceType{6}  DevicePara=DevicePara{6}  PowerFlow=DevicePowerFlow{6}  x0=x_e{6}  OtherInputs=OtherInputs{6}  DiscreMethod=Hybrid Trapezoidal  EnableInsideModification=off  DiscreDampingFlag=on  DiscreDampingValue=DeviceDiscreDamping{6}  LinearizationTimes=1  DirectFeedthrough=off
  SM7 : SimplexPS/Synchronous Machine (dq-Frame System Object)  Ts=Ts  Sbase=Sbase  Vbase=Vbase  Wbase=Wbase  DeviceType=DeviceType{7}  DevicePara=DevicePara{7}  PowerFlow=DevicePowerFlow{7}  x0=x_e{7}  OtherInputs=OtherInputs{7}  DiscreMethod=Hybrid Trapezoidal  EnableInsideModification=off  DiscreDampingFlag=on  DiscreDampingValue=DeviceDiscreDamping{7}  LinearizationTimes=1  DirectFeedthrough=off
  SM8 : SimplexPS/Synchronous Machine (dq-Frame System Object)  Ts=Ts  Sbase=Sbase  Vbase=Vbase  Wbase=Wbase  DeviceType=DeviceType{8}  DevicePara=DevicePara{8}  PowerFlow=DevicePowerFlow{8}  x0=x_e{8}  OtherInputs=OtherInputs{8}  DiscreMethod=Hybrid Trapezoidal  EnableInsideModification=off  DiscreDampingFlag=on  DiscreDampingValue=DeviceDiscreDamping{8}  LinearizationTimes=1  DirectFeedthrough=off
  SM9 : SimplexPS/Synchronous Machine (dq-Frame System Object)  Ts=Ts  Sbase=Sbase  Vbase=Vbase  Wbase=Wbase  DeviceType=DeviceType{9}  DevicePara=DevicePara{9}  PowerFlow=DevicePowerFlow{9}  x0=x_e{9}  OtherInputs=OtherInputs{9}  DiscreMethod=Hybrid Trapezoidal  EnableInsideModification=off  DiscreDampingFlag=on  DiscreDampingValue=DeviceDiscreDamping{9}  LinearizationTimes=1  DirectFeedthrough=off
  Scope1 : Scope
  Transformer10-31 : powerlib/Elements/Three-Phase Transformer (Two Windings)  Winding1Connection=Yg  Winding2Connection=Yg  CoreType=Three single-phase transformers  SetSaturation=off  Hysteresis=off  DataFile='hysteresis'  SetInitialFlux=off  Measurements=None  UNITS=pu  NominalPower=[Sbase, Fbase]  Winding1=[1.04*Vbase, 0, 0]  Winding2=[Vbase, 0, 0]  Rm=1e4  Lm=1e4  L0=0.5  Saturation=[ 0,0 ; 0.0024,1.2 ; 1.0,1.52 ]  InitialFluxes=[ 0.8 , -0.8 , 0.7 ]  BreakLoop=off  DiscreteSolver=Trapezoidal iterative  DataType=off  TransfoNumber=1
  Transformer11-32 : powerlib/Elements/Three-Phase Transformer (Two Windings)  Winding1Connection=Yg  Winding2Connection=Yg  CoreType=Three single-phase transformers  SetSaturation=off  Hysteresis=off  DataFile='hysteresis'  SetInitialFlux=off  Measurements=None  UNITS=pu  NominalPower=[Sbase, Fbase]  Winding1=[1.04*Vbase, 0, 0]  Winding2=[Vbase, 0, 0]  Rm=1e4  Lm=1e4  L0=0.5  Saturation=[ 0,0 ; 0.0024,1.2 ; 1.0,1.52 ]  InitialFluxes=[ 0.8 , -0.8 , 0.7 ]  BreakLoop=off  DiscreteSolver=Trapezoidal iterative  DataType=off  TransfoNumber=1
  Transformer12-36 : powerlib/Elements/Three-Phase Transformer (Two Windings)  Winding1Connection=Yg  Winding2Connection=Yg  CoreType=Three single-phase transformers  SetSaturation=off  Hysteresis=off  DataFile='hysteresis'  SetInitialFlux=off  Measurements=None  UNITS=pu  NominalPower=[Sbase, Fbase]  Winding1=[1.04*Vbase, 0, 0]  Winding2=[Vbase, 0, 0]  Rm=1e4  Lm=1e4  L0=0.5  Saturation=[ 0,0 ; 0.0024,1.2 ; 1.0,1.52 ]  InitialFluxes=[ 0.8 , -0.8 , 0.7 ]  BreakLoop=off  DiscreteSolver=Trapezoidal iterative  DataType=off  TransfoNumber=1
  Transformer13-17 : powerlib/Elements/Three-Phase Transformer (Two Windings)  Winding1Connection=Yg  Winding2Connection=Yg  CoreType=Three single-phase transformers  SetSaturation=off  Hysteresis=off  DataFile='hysteresis'  SetInitialFlux=off  Measurements=None  UNITS=pu  NominalPower=[Sbase, Fbase]  Winding1=[1.04*Vbase, 0, 0]  Winding2=[Vbase, 0, 0]  Rm=1e4  Lm=1e4  L0=0.5  Saturation=[ 0,0 ; 0.0024,1.2 ; 1.0,1.52 ]  InitialFluxes=[ 0.8 , -0.8 , 0.7 ]  BreakLoop=off  DiscreteSolver=Trapezoidal iterative  DataType=off  TransfoNumber=1
  Transformer16-54 : powerlib/Elements/Three-Phase Transformer (Two Windings)  Winding1Connection=Yg  Winding2Connection=Yg  CoreType=Three single-phase transformers  SetSaturation=off  Hysteresis=off  DataFile='hysteresis'  SetInitialFlux=off  Measurements=None  UNITS=pu  NominalPower=[Sbase, Fbase]  Winding1=[1.025*Vbase, 0, 0]  Winding2=[Vbase, 0, 0]  Rm=1e4  Lm=1e4  L0=0.5  Saturation=[ 0,0 ; 0.0024,1.2 ; 1.0,1.52 ]  InitialFluxes=[ 0.8 , -0.8 , 0.7 ]  BreakLoop=off  DiscreteSolver=Trapezoidal iterative  DataType=off  TransfoNumber=1
  Transformer19-20 : powerlib/Elements/Three-Phase Transformer (Two Windings)  Winding1Connection=Yg  Winding2Connection=Yg  CoreType=Three single-phase transformers  SetSaturation=off  Hysteresis=off  DataFile='hysteresis'  SetInitialFlux=off  Measurements=None  UNITS=pu  NominalPower=[Sbase, Fbase]  Winding1=[0.9434*Vbase, 0, 0]  Winding2=[Vbase, 0, 0]  Rm=1e4  Lm=1e4  L0=0.5  Saturation=[ 0,0 ; 0.0024,1.2 ; 1.0,1.52 ]  InitialFluxes=[ 0.8 , -0.8 , 0.7 ]  BreakLoop=off  DiscreteSolver=Trapezoidal iterative  DataType=off  TransfoNumber=1
  Transformer2-58 : powerlib/Elements/Three-Phase Transformer (Two Windings)  Winding1Connection=Yg  Winding2Connection=Yg  CoreType=Three single-phase transformers  SetSaturation=off  Hysteresis=off  DataFile='hysteresis'  SetInitialFlux=off  Measurements=None  UNITS=pu  NominalPower=[Sbase, Fbase]  Winding1=[1.07*Vbase, 0, 0]  Winding2=[Vbase, 0, 0]  Rm=1e4  Lm=1e4  L0=0.5  Saturation=[ 0,0 ; 0.0024,1.2 ; 1.0,1.52 ]  InitialFluxes=[ 0.8 , -0.8 , 0.7 ]  BreakLoop=off  DiscreteSolver=Trapezoidal iterative  DataType=off  TransfoNumber=1
  Transformer3-62 : powerlib/Elements/Three-Phase Transformer (Two Windings)  Winding1Connection=Yg  Winding2Connection=Yg  CoreType=Three single-phase transformers  SetSaturation=off  Hysteresis=off  DataFile='hysteresis'  SetInitialFlux=off  Measurements=None  UNITS=pu  NominalPower=[Sbase, Fbase]  Winding1=[1.07*Vbase, 0, 0]  Winding2=[Vbase, 0, 0]  Rm=1e4  Lm=1e4  L0=0.5  Saturation=[ 0,0 ; 0.0024,1.2 ; 1.0,1.52 ]  InitialFluxes=[ 0.8 , -0.8 , 0.7 ]  BreakLoop=off  DiscreteSolver=Trapezoidal iterative  DataType=off  TransfoNumber=1
  Transformer34-35 : powerlib/Elements/Three-Phase Transformer (Two Windings)  Winding1Connection=Yg  Winding2Connection=Yg  CoreType=Three single-phase transformers  SetSaturation=off  Hysteresis=off  DataFile='hysteresis'  SetInitialFlux=off  Measurements=None  UNITS=pu  NominalPower=[Sbase, Fbase]  Winding1=[0.946*Vbase, 0, 0]  Winding2=[Vbase, 0, 0]  Rm=1e4  Lm=1e4  L0=0.5  Saturation=[ 0,0 ; 0.0024,1.2 ; 1.0,1.52 ]  InitialFluxes=[ 0.8 , -0.8 , 0.7 ]  BreakLoop=off  DiscreteSolver=Trapezoidal iterative  DataType=off  TransfoNumber=1
  Transformer4-19 : powerlib/Elements/Three-Phase Transformer (Two Windings)  Winding1Connection=Yg  Winding2Connection=Yg  CoreType=Three single-phase transformers  SetSaturation=off  Hysteresis=off  DataFile='hysteresis'  SetInitialFlux=off  Measurements=None  UNITS=pu  NominalPower=[Sbase, Fbase]  Winding1=[1.07*Vbase, 0, 0]  Winding2=[Vbase, 0, 0]  Rm=1e4  Lm=1e4  L0=0.5  Saturation=[ 0,0 ; 0.0024,1.2 ; 1.0,1.52 ]  InitialFluxes=[ 0.8 , -0.8 , 0.7 ]  BreakLoop=off  DiscreteSolver=Trapezoidal iterative  DataType=off  TransfoNumber=1
  Transformer5-20 : powerlib/Elements/Three-Phase Transformer (Two Windings)  Winding1Connection=Yg  Winding2Connection=Yg  CoreType=Three single-phase transformers  SetSaturation=off  Hysteresis=off  DataFile='hysteresis'  SetInitialFlux=off  Measurements=None  UNITS=pu  NominalPower=[Sbase, Fbase]  Winding1=[1.009*Vbase, 0, 0]  Winding2=[Vbase, 0, 0]  Rm=1e4  Lm=1e4  L0=0.5  Saturation=[ 0,0 ; 0.0024,1.2 ; 1.0,1.52 ]  InitialFluxes=[ 0.8 , -0.8 , 0.7 ]  BreakLoop=off  DiscreteSolver=Trapezoidal iterative  DataType=off  TransfoNumber=1
  Transformer6-22 : powerlib/Elements/Three-Phase Transformer (Two Windings)  Winding1Connection=Yg  Winding2Connection=Yg  CoreType=Three single-phase transformers  SetSaturation=off  Hysteresis=off  DataFile='hysteresis'  SetInitialFlux=off  Measurements=None  UNITS=pu  NominalPower=[Sbase, Fbase]  Winding1=[1.025*Vbase, 0, 0]  Winding2=[Vbase, 0, 0]  Rm=1e4  Lm=1e4  L0=0.5  Saturation=[ 0,0 ; 0.0024,1.2 ; 1.0,1.52 ]  InitialFluxes=[ 0.8 , -0.8 , 0.7 ]  BreakLoop=off  DiscreteSolver=Trapezoidal iterative  DataType=off  TransfoNumber=1
  Transformer63-64 : powerlib/Elements/Three-Phase Transformer (Two Windings)  Winding1Connection=Yg  Winding2Connection=Yg  CoreType=Three single-phase transformers  SetSaturation=off  Hysteresis=off  DataFile='hysteresis'  SetInitialFlux=off  Measurements=None  UNITS=pu  NominalPower=[Sbase, Fbase]  Winding1=[1.06*Vbase, 0, 0]  Winding2=[Vbase, 0, 0]  Rm=1e4  Lm=1e4  L0=0.5  Saturation=[ 0,0 ; 0.0024,1.2 ; 1.0,1.52 ]  InitialFluxes=[ 0.8 , -0.8 , 0.7 ]  BreakLoop=off  DiscreteSolver=Trapezoidal iterative  DataType=off  TransfoNumber=1
  Transformer64-65 : powerlib/Elements/Three-Phase Transformer (Two Windings)  Winding1Connection=Yg  Winding2Connection=Yg  CoreType=Three single-phase transformers  SetSaturation=off  Hysteresis=off  DataFile='hysteresis'  SetInitialFlux=off  Measurements=None  UNITS=pu  NominalPower=[Sbase, Fbase]  Winding1=[0.9434*Vbase, 0, 0]  Winding2=[Vbase, 0, 0]  Rm=1e4  Lm=1e4  L0=0.5  Saturation=[ 0,0 ; 0.0024,1.2 ; 1.0,1.52 ]  InitialFluxes=[ 0.8 , -0.8 , 0.7 ]  BreakLoop=off  DiscreteSolver=Trapezoidal iterative  DataType=off  TransfoNumber=1
  Transformer8-25 : powerlib/Elements/Three-Phase Transformer (Two Windings)  Winding1Connection=Yg  Winding2Connection=Yg  CoreType=Three single-phase transformers  SetSaturation=off  Hysteresis=off  DataFile='hysteresis'  SetInitialFlux=off  Measurements=None  UNITS=pu  NominalPower=[Sbase, Fbase]  Winding1=[1.025*Vbase, 0, 0]  Winding2=[Vbase, 0, 0]  Rm=1e4  Lm=1e4  L0=0.5  Saturation=[ 0,0 ; 0.0024,1.2 ; 1.0,1.52 ]  InitialFluxes=[ 0.8 , -0.8 , 0.7 ]  BreakLoop=off  DiscreteSolver=Trapezoidal iterative  DataType=off  TransfoNumber=1
  Transformer9-29 : powerlib/Elements/Three-Phase Transformer (Two Windings)  Winding1Connection=Yg  Winding2Connection=Yg  CoreType=Three single-phase transformers  SetSaturation=off  Hysteresis=off  DataFile='hysteresis'  SetInitialFlux=off  Measurements=None  UNITS=pu  NominalPower=[Sbase, Fbase]  Winding1=[1.025*Vbase, 0, 0]  Winding2=[Vbase, 0, 0]  Rm=1e4  Lm=1e4  L0=0.5  Saturation=[ 0,0 ; 0.0024,1.2 ; 1.0,1.52 ]  InitialFluxes=[ 0.8 , -0.8 , 0.7 ]  BreakLoop=off  DiscreteSolver=Trapezoidal iterative  DataType=off  TransfoNumber=1
  powergui : powerlib/powergui  Priority=1  SimulationMode=Discrete  SampleTime=Ts  frequency=60  Iterations=50  frequencyindice=0  Pbase=100e6  ErrMax=1e-4  UnitsV=kV  UnitsW=MW  buscounter=0  FunctionMessages=off  echomessages=off  EnableUseOfTLC=off  CurrentSourceSwitches=off  DisableSnubberDevices=off  DisableRonSwitches=off  DisableVfSwitches=off  DisplayEquations=off  AutomaticDiscreteSolvers=off  SolverType=Tustin/Backward Euler (TBE)  Interpol=off  ExternalGateDelay=off  methode=off  Ts=100  x0status=blocks  SPID=on  SwTol=0  HookPort=off  NonlinearTolerance=1e-4  nMaxIteration=100  ContinueOnMaxIteration=off  RestoreLinks=warning  ResistiveCurrentMeasurement=off  Frange=[0:2:500]  Ylog=off  Xlog=on  ShowGrid=off  save=off  variable=ZData  structure=0  ZoomFFT=off  StartTime=0.0  cycles=1  DisplayStyle=1  fundamental=60  FreqAxis=off  MaxFrequency=1000  frequencyindicesteady=1  RmsSteady=1  display=off
  wires:
  SM1/1 -> DS-Bus1/1
  DS-Bus1/1 -> D-Scope1/1  "<v_dq>"
  DS-Bus1/2 -> D-Scope1/2  "<i_dq>"
  DS-Bus1/3 -> D-Scope1/3  "<v_abc>"
  DS-Bus1/4 -> D-Scope1/4  "<i_abc>"
  DS-Bus1/5 -> D-Scope1/5  "<w>"
  DS-Bus1/6 -> D-Scope1/6  "<theta>"
  DS-Bus1/7 -> D-Scope1/7  "<pq>"
  SM2/1 -> DS-Bus2/1
  DS-Bus2/1 -> D-Scope2/1  "<v_dq>"
  DS-Bus2/2 -> D-Scope2/2  "<i_dq>"
  DS-Bus2/3 -> D-Scope2/3  "<v_abc>"
  DS-Bus2/4 -> D-Scope2/4  "<i_abc>"
  DS-Bus2/5 -> D-Scope2/5  "<w>"
  DS-Bus2/6 -> D-Scope2/6  "<theta>"
  DS-Bus2/7 -> D-Scope2/7  "<pq>"
  SM3/1 -> DS-Bus3/1
  DS-Bus3/1 -> D-Scope3/1  "<v_dq>"
  DS-Bus3/2 -> D-Scope3/2  "<i_dq>"
  DS-Bus3/3 -> D-Scope3/3  "<v_abc>"
  DS-Bus3/4 -> D-Scope3/4  "<i_abc>"
  DS-Bus3/5 -> D-Scope3/5  "<w>"
  DS-Bus3/6 -> D-Scope3/6  "<theta>"
  DS-Bus3/7 -> D-Scope3/7  "<pq>"
  SM4/1 -> DS-Bus4/1
  DS-Bus4/1 -> D-Scope4/1  "<v_dq>"
  DS-Bus4/2 -> D-Scope4/2  "<i_dq>"
  DS-Bus4/3 -> D-Scope4/3  "<v_abc>"
  DS-Bus4/4 -> D-Scope4/4  "<i_abc>"
  DS-Bus4/5 -> D-Scope4/5  "<w>"
  DS-Bus4/6 -> D-Scope4/6  "<theta>"
  DS-Bus4/7 -> D-Scope4/7  "<pq>"
  SM5/1 -> DS-Bus5/1
  DS-Bus5/1 -> D-Scope5/1  "<v_dq>"
  DS-Bus5/2 -> D-Scope5/2  "<i_dq>"
  DS-Bus5/3 -> D-Scope5/3  "<v_abc>"
  DS-Bus5/4 -> D-Scope5/4  "<i_abc>"
  DS-Bus5/5 -> D-Scope5/5  "<w>"
  DS-Bus5/6 -> D-Scope5/6  "<theta>"
  DS-Bus5/7 -> D-Scope5/7  "<pq>"
  SM6/1 -> DS-Bus6/1
  DS-Bus6/1 -> D-Scope6/1  "<v_dq>"
  DS-Bus6/2 -> D-Scope6/2  "<i_dq>"
  DS-Bus6/3 -> D-Scope6/3  "<v_abc>"
  DS-Bus6/4 -> D-Scope6/4  "<i_abc>"
  DS-Bus6/5 -> D-Scope6/5  "<w>"
  DS-Bus6/6 -> D-Scope6/6  "<theta>"
  DS-Bus6/7 -> D-Scope6/7  "<pq>"
  SM7/1 -> DS-Bus7/1
  DS-Bus7/1 -> D-Scope7/1  "<v_dq>"
  DS-Bus7/2 -> D-Scope7/2  "<i_dq>"
  DS-Bus7/3 -> D-Scope7/3  "<v_abc>"
  DS-Bus7/4 -> D-Scope7/4  "<i_abc>"
  DS-Bus7/5 -> D-Scope7/5  "<w>"
  DS-Bus7/6 -> D-Scope7/6  "<theta>"
  DS-Bus7/7 -> D-Scope7/7  "<pq>"
  SM8/1 -> DS-Bus8/1
  DS-Bus8/1 -> D-Scope8/1  "<v_dq>"
  DS-Bus8/2 -> D-Scope8/2  "<i_dq>"
  DS-Bus8/3 -> D-Scope8/3  "<v_abc>"
  DS-Bus8/4 -> D-Scope8/4  "<i_abc>"
  DS-Bus8/5 -> D-Scope8/5  "<w>"
  DS-Bus8/6 -> D-Scope8/6  "<theta>"
  DS-Bus8/7 -> D-Scope8/7  "<pq>"
  SM9/1 -> DS-Bus9/1
  DS-Bus9/1 -> D-Scope9/1  "<v_dq>"
  DS-Bus9/2 -> D-Scope9/2  "<i_dq>"
  DS-Bus9/3 -> D-Scope9/3  "<v_abc>"
  DS-Bus9/4 -> D-Scope9/4  "<i_abc>"
  DS-Bus9/5 -> D-Scope9/5  "<w>"
  DS-Bus9/6 -> D-Scope9/6  "<theta>"
  DS-Bus9/7 -> D-Scope9/7  "<pq>"
  SM10/1 -> DS-Bus10/1
  DS-Bus10/1 -> D-Scope10/1  "<v_dq>"
  DS-Bus10/2 -> D-Scope10/2  "<i_dq>"
  DS-Bus10/3 -> D-Scope10/3  "<v_abc>"
  DS-Bus10/4 -> D-Scope10/4  "<i_abc>"
  DS-Bus10/5 -> D-Scope10/5  "<w>"
  DS-Bus10/6 -> D-Scope10/6  "<theta>"
  DS-Bus10/7 -> D-Scope10/7  "<pq>"
  SM11/1 -> DS-Bus11/1
  DS-Bus11/1 -> D-Scope11/1  "<v_dq>"
  DS-Bus11/2 -> D-Scope11/2  "<i_dq>"
  DS-Bus11/3 -> D-Scope11/3  "<v_abc>"
  DS-Bus11/4 -> D-Scope11/4  "<i_abc>"
  DS-Bus11/5 -> D-Scope11/5  "<w>"
  DS-Bus11/6 -> D-Scope11/6  "<theta>"
  DS-Bus11/7 -> D-Scope11/7  "<pq>"
  SM12/1 -> DS-Bus12/1
  DS-Bus12/1 -> D-Scope12/1  "<v_dq>"
  DS-Bus12/2 -> D-Scope12/2  "<i_dq>"
  DS-Bus12/3 -> D-Scope12/3  "<v_abc>"
  DS-Bus12/4 -> D-Scope12/4  "<i_abc>"
  DS-Bus12/5 -> D-Scope12/5  "<w>"
  DS-Bus12/6 -> D-Scope12/6  "<theta>"
  DS-Bus12/7 -> D-Scope12/7  "<pq>"
  SM13/1 -> DS-Bus13/1
  DS-Bus13/1 -> D-Scope13/1  "<v_dq>"
  DS-Bus13/2 -> D-Scope13/2  "<i_dq>"
  DS-Bus13/3 -> D-Scope13/3  "<v_abc>"
  DS-Bus13/4 -> D-Scope13/4  "<i_abc>"
  DS-Bus13/5 -> D-Scope13/5  "<w>"
  DS-Bus13/6 -> D-Scope13/6  "<theta>"
  DS-Bus13/7 -> D-Scope13/7  "<pq>"
  SM14/1 -> DS-Bus14/1
  DS-Bus14/1 -> D-Scope14/1  "<v_dq>"
  DS-Bus14/2 -> D-Scope14/2  "<i_dq>"
  DS-Bus14/3 -> D-Scope14/3  "<v_abc>"
  DS-Bus14/4 -> D-Scope14/4  "<i_abc>"
  DS-Bus14/5 -> D-Scope14/5  "<w>"
  DS-Bus14/6 -> D-Scope14/6  "<theta>"
  DS-Bus14/7 -> D-Scope14/7  "<pq>"
  SM15/1 -> DS-Bus15/1
  DS-Bus15/1 -> D-Scope15/1  "<v_dq>"
  DS-Bus15/2 -> D-Scope15/2  "<i_dq>"
  DS-Bus15/3 -> D-Scope15/3  "<v_abc>"
  DS-Bus15/4 -> D-Scope15/4  "<i_abc>"
  DS-Bus15/5 -> D-Scope15/5  "<w>"
  DS-Bus15/6 -> D-Scope15/6  "<theta>"
  DS-Bus15/7 -> D-Scope15/7  "<pq>"
  SM16/1 -> DS-Bus16/1
  DS-Bus16/1 -> D-Scope16/1  "<v_dq>"
  DS-Bus16/2 -> D-Scope16/2  "<i_dq>"
  DS-Bus16/3 -> D-Scope16/3  "<v_abc>"
  DS-Bus16/4 -> D-Scope16/4  "<i_abc>"
  DS-Bus16/5 -> D-Scope16/5  "<w>"
  DS-Bus16/6 -> D-Scope16/6  "<theta>"
  DS-Bus16/7 -> D-Scope16/7  "<pq>"
  Current Measurement1/1 -> Scope1/1
  connections:
  SM1/LConn4 -- D-GND1/LConn1
  SM2/LConn4 -- D-GND2/LConn1
  SM3/LConn4 -- D-GND3/LConn1
  SM4/LConn4 -- D-GND4/LConn1
  SM5/LConn4 -- D-GND5/LConn1
  SM6/LConn4 -- D-GND6/LConn1
  SM7/LConn4 -- D-GND7/LConn1
  SM8/LConn4 -- D-GND8/LConn1
  SM9/LConn4 -- D-GND9/LConn1
  SM10/LConn4 -- D-GND10/LConn1
  SM11/LConn4 -- D-GND11/LConn1
  SM12/LConn4 -- D-GND12/LConn1
  SM13/LConn4 -- D-GND13/LConn1
  SM14/LConn4 -- D-GND14/LConn1
  SM15/LConn4 -- D-GND15/LConn1
  SM16/LConn4 -- D-GND16/LConn1
  Branch17-17/RConn1 -- Branch17-17/RConn2 -- Branch17-17/RConn3 -- B-GND17/LConn1
  Branch18-18/RConn1 -- Branch18-18/RConn2 -- Branch18-18/RConn3 -- B-GND20/LConn1
  Branch19-19/RConn1 -- Branch19-19/RConn2 -- Branch19-19/RConn3 -- B-GND24/LConn1
  Branch20-20/RConn1 -- Branch20-20/RConn2 -- Branch20-20/RConn3 -- B-GND27/LConn1
  Branch21-21/RConn1 -- Branch21-21/RConn2 -- Branch21-21/RConn3 -- B-GND28/LConn1
  Branch22-22/RConn1 -- Branch22-22/RConn2 -- Branch22-22/RConn3 -- B-GND31/LConn1
  Branch23-23/RConn1 -- Branch23-23/RConn2 -- Branch23-23/RConn3 -- B-GND33/LConn1
  Branch24-24/RConn1 -- Branch24-24/RConn2 -- Branch24-24/RConn3 -- B-GND35/LConn1
  Branch25-25/RConn1 -- Branch25-25/RConn2 -- Branch25-25/RConn3 -- B-GND37/LConn1
  Branch26-26/RConn1 -- Branch26-26/RConn2 -- Branch26-26/RConn3 -- B-GND40/LConn1
  Branch27-27/RConn1 -- Branch27-27/RConn2 -- Branch27-27/RConn3 -- B-GND44/LConn1
  Branch28-28/RConn1 -- Branch28-28/RConn2 -- Branch28-28/RConn3 -- B-GND47/LConn1
  Branch29-29/RConn1 -- Branch29-29/RConn2 -- Branch29-29/RConn3 -- B-GND49/LConn1
  Branch30-30/RConn1 -- Branch30-30/RConn2 -- Branch30-30/RConn3 -- B-GND50/LConn1
  Branch31-31/RConn1 -- Branch31-31/RConn2 -- Branch31-31/RConn3 -- B-GND55/LConn1
  Branch32-32/RConn1 -- Branch32-32/RConn2 -- Branch32-32/RConn3 -- B-GND58/LConn1
  Branch33-33/RConn1 -- Branch33-33/RConn2 -- Branch33-33/RConn3 -- B-GND60/LConn1
  Branch34-34/RConn1 -- Branch34-34/RConn2 -- Branch34-34/RConn3 -- B-GND63/LConn1
  Branch35-35/RConn1 -- Branch35-35/RConn2 -- Branch35-35/RConn3 -- B-GND66/LConn1
  Branch36-36/RConn1 -- Branch36-36/RConn2 -- Branch36-36/RConn3 -- B-GND68/LConn1
  Branch37-37/RConn1 -- Branch37-37/RConn2 -- Branch37-37/RConn3 -- B-GND70/LConn1
  Branch38-38/RConn1 -- Branch38-38/RConn2 -- Branch38-38/RConn3 -- B-GND73/LConn1
  Branch39-39/RConn1 -- Branch39-39/RConn2 -- Branch39-39/RConn3 -- B-GND75/LConn1
  Branch40-40/RConn1 -- Branch40-40/RConn2 -- Branch40-40/RConn3 -- B-GND78/LConn1
  Branch41-41/RConn1 -- Branch41-41/RConn2 -- Branch41-41/RConn3 -- B-GND81/LConn1
  Branch42-42/RConn1 -- Branch42-42/RConn2 -- Branch42-42/RConn3 -- B-GND83/LConn1
  Branch44-44/RConn1 -- Branch44-44/RConn2 -- Branch44-44/RConn3 -- B-GND85/LConn1
  Branch45-45/RConn1 -- Branch45-45/RConn2 -- Branch45-45/RConn3 -- B-GND87/LConn1
  Branch46-46/RConn1 -- Branch46-46/RConn2 -- Branch46-46/RConn3 -- B-GND89/LConn1
  Branch47-47/RConn1 -- Branch47-47/RConn2 -- Branch47-47/RConn3 -- B-GND91/LConn1
  Branch48-48/RConn1 -- Branch48-48/RConn2 -- Branch48-48/RConn3 -- B-GND94/LConn1
  Branch49-49/RConn1 -- Branch49-49/RConn2 -- Branch49-49/RConn3 -- B-GND95/LConn1
  Branch50-50/RConn1 -- Branch50-50/RConn2 -- Branch50-50/RConn3 -- B-GND96/LConn1
  Branch51-51/RConn1 -- Branch51-51/RConn2 -- Branch51-51/RConn3 -- B-GND98/LConn1
  Branch52-52/RConn1 -- Branch52-52/RConn2 -- Branch52-52/RConn3 -- B-GND99/LConn1
  Branch53-53/RConn1 -- Branch53-53/RConn2 -- Branch53-53/RConn3 -- B-GND101/LConn1
  Branch54-54/RConn1 -- Branch54-54/RConn2 -- Branch54-54/RConn3 -- B-GND103/LConn1
  Branch55-55/RConn1 -- Branch55-55/RConn2 -- Branch55-55/RConn3 -- B-GND105/LConn1
  Branch56-56/RConn1 -- Branch56-56/RConn2 -- Branch56-56/RConn3 -- B-GND107/LConn1
  Branch57-57/RConn1 -- Branch57-57/RConn2 -- Branch57-57/RConn3 -- B-GND110/LConn1
  Branch58-58/RConn1 -- Branch58-58/RConn2 -- Branch58-58/RConn3 -- B-GND113/LConn1
  Branch59-59/RConn1 -- Branch59-59/RConn2 -- Branch59-59/RConn3 -- B-GND116/LConn1
  Branch60-60/RConn1 -- Branch60-60/RConn2 -- Branch60-60/RConn3 -- B-GND118/LConn1
  Branch61-61/RConn1 -- Branch61-61/RConn2 -- Branch61-61/RConn3 -- B-GND120/LConn1
  Branch62-62/RConn1 -- Branch62-62/RConn2 -- Branch62-62/RConn3 -- B-GND121/LConn1
  Branch63-63/RConn1 -- Branch63-63/RConn2 -- Branch63-63/RConn3 -- B-GND124/LConn1
  Branch64-64/RConn1 -- Branch64-64/RConn2 -- Branch64-64/RConn3 -- B-GND126/LConn1
  Branch65-65/RConn1 -- Branch65-65/RConn2 -- Branch65-65/RConn3 -- B-GND128/LConn1
  Branch66-66/RConn1 -- Branch66-66/RConn2 -- Branch66-66/RConn3 -- B-GND130/LConn1
  Branch67-67/RConn1 -- Branch67-67/RConn2 -- Branch67-67/RConn3 -- B-GND132/LConn1
  Branch68-68/RConn1 -- Branch68-68/RConn2 -- Branch68-68/RConn3 -- B-GND134/LConn1
  Branch1-18/RConn1 -- Bus18/RConn1 -- Branch18-18/LConn1 -- Branch18-50/LConn1 -- Branch18-49/LConn1 -- Branch18-42/LConn1
  Branch1-18/RConn2 -- Bus18/RConn2 -- Branch18-18/LConn2 -- Branch18-50/LConn2 -- Branch18-49/LConn2 -- Branch18-42/LConn2
  Branch1-18/RConn3 -- Bus18/RConn3 -- Branch18-18/LConn3 -- Branch18-50/LConn3 -- Branch18-49/LConn3 -- Branch18-42/LConn3
  Bus1/RConn1 -- Branch1-18/LConn1
  Bus1/RConn2 -- Branch1-18/LConn2
  Bus1/RConn3 -- Branch1-18/LConn3
  Branch2-58/RConn1 -- Bus58/RConn1 -- Branch58-58/LConn1 -- Branch58-63/LConn1 -- Branch58-59/LConn1 -- Branch57-58/RConn1
  Branch2-58/RConn2 -- Bus58/RConn2 -- Branch58-58/LConn2 -- Branch58-63/LConn2 -- Branch58-59/LConn2 -- Branch57-58/RConn2
  Branch2-58/RConn3 -- Bus58/RConn3 -- Branch58-58/LConn3 -- Branch58-63/LConn3 -- Branch58-59/LConn3 -- Branch57-58/RConn3
  Transformer2-58/RConn1 -- Branch2-58/LConn1
  Transformer2-58/RConn2 -- Branch2-58/LConn2
  Transformer2-58/RConn3 -- Branch2-58/LConn3
  Bus2/RConn1 -- Transformer2-58/LConn1
  Bus2/RConn2 -- Transformer2-58/LConn2
  Bus2/RConn3 -- Transformer2-58/LConn3
  Branch3-62/RConn1 -- Bus62/RConn1 -- Branch62-62/LConn1 -- Branch62-65/LConn1 -- Branch62-63/LConn1
  Branch3-62/RConn2 -- Bus62/RConn2 -- Branch62-62/LConn2 -- Branch62-65/LConn2 -- Branch62-63/LConn2
  Branch3-62/RConn3 -- Bus62/RConn3 -- Branch62-62/LConn3 -- Branch62-65/LConn3 -- Branch62-63/LConn3
  Transformer3-62/RConn1 -- Branch3-62/LConn1
  Transformer3-62/RConn2 -- Branch3-62/LConn2
  Transformer3-62/RConn3 -- Branch3-62/LConn3
  Bus3/RConn1 -- Transformer3-62/LConn1
  Bus3/RConn2 -- Transformer3-62/LConn2
  Bus3/RConn3 -- Transformer3-62/LConn3
  Branch4-19/RConn1 -- Bus19/RConn1 -- Branch19-19/LConn1 -- Branch19-68/LConn1 -- Transformer19-20/LConn1
  Branch4-19/RConn2 -- Bus19/RConn2 -- Branch19-19/LConn2 -- Branch19-68/LConn2 -- Transformer19-20/LConn2
  Branch4-19/RConn3 -- Bus19/RConn3 -- Branch19-19/LConn3 -- Branch19-68/LConn3 -- Transformer19-20/LConn3
  Transformer4-19/RConn1 -- Branch4-19/LConn1
  Transformer4-19/RConn2 -- Branch4-19/LConn2
  Transformer4-19/RConn3 -- Branch4-19/LConn3
  Bus4/RConn1 -- Transformer4-19/LConn1
  Bus4/RConn2 -- Transformer4-19/LConn2
  Bus4/RConn3 -- Transformer4-19/LConn3
  Branch5-20/RConn1 -- Bus20/RConn1 -- Branch20-20/LConn1 -- Branch19-20/RConn1
  Branch5-20/RConn2 -- Bus20/RConn2 -- Branch20-20/LConn2 -- Branch19-20/RConn2
  Branch5-20/RConn3 -- Bus20/RConn3 -- Branch20-20/LConn3 -- Branch19-20/RConn3
  Transformer5-20/RConn1 -- Branch5-20/LConn1
  Transformer5-20/RConn2 -- Branch5-20/LConn2
  Transformer5-20/RConn3 -- Branch5-20/LConn3
  Bus5/RConn1 -- Transformer5-20/LConn1
  Bus5/RConn2 -- Transformer5-20/LConn2
  Bus5/RConn3 -- Transformer5-20/LConn3
  Branch6-22/RConn1 -- Bus22/RConn1 -- Branch22-22/LConn1 -- Branch22-23/LConn1 -- Branch21-22/RConn1
  Branch6-22/RConn2 -- Bus22/RConn2 -- Branch22-22/LConn2 -- Branch22-23/LConn2 -- Branch21-22/RConn2
  Branch6-22/RConn3 -- Bus22/RConn3 -- Branch22-22/LConn3 -- Branch22-23/LConn3 -- Branch21-22/RConn3
  Transformer6-22/RConn1 -- Branch6-22/LConn1
  Transformer6-22/RConn2 -- Branch6-22/LConn2
  Transformer6-22/RConn3 -- Branch6-22/LConn3
  Bus6/RConn1 -- Transformer6-22/LConn1
  Bus6/RConn2 -- Transformer6-22/LConn2
  Bus6/RConn3 -- Transformer6-22/LConn3
  Branch7-23/RConn1 -- Bus23/RConn1 -- Branch23-23/LConn1 -- Branch23-24/LConn1 -- Branch22-23/RConn1
  Branch7-23/RConn2 -- Bus23/RConn2 -- Branch23-23/LConn2 -- Branch23-24/LConn2 -- Branch22-23/RConn2
  Branch7-23/RConn3 -- Bus23/RConn3 -- Branch23-23/LConn3 -- Branch23-24/LConn3 -- Branch22-23/RConn3
  Bus7/RConn1 -- Branch7-23/LConn1
  Bus7/RConn2 -- Branch7-23/LConn2
  Bus7/RConn3 -- Branch7-23/LConn3
  Branch8-25/RConn1 -- Bus25/RConn1 -- Branch25-25/LConn1 -- Branch25-54/LConn1 -- Branch25-26/LConn1
  Branch8-25/RConn2 -- Bus25/RConn2 -- Branch25-25/LConn2 -- Branch25-54/LConn2 -- Branch25-26/LConn2
  Branch8-25/RConn3 -- Bus25/RConn3 -- Branch25-25/LConn3 -- Branch25-54/LConn3 -- Branch25-26/LConn3
  Transformer8-25/RConn1 -- Branch8-25/LConn1
  Transformer8-25/RConn2 -- Branch8-25/LConn2
  Transformer8-25/RConn3 -- Branch8-25/LConn3
  Bus8/RConn1 -- Transformer8-25/LConn1
  Bus8/RConn2 -- Transformer8-25/LConn2
  Bus8/RConn3 -- Transformer8-25/LConn3
  Branch9-29/RConn1 -- Bus29/RConn1 -- Branch29-29/LConn1 -- Branch28-29/RConn1 -- Branch26-29/RConn1
  Branch9-29/RConn2 -- Bus29/RConn2 -- Branch29-29/LConn2 -- Branch28-29/RConn2 -- Branch26-29/RConn2
  Branch9-29/RConn3 -- Bus29/RConn3 -- Branch29-29/LConn3 -- Branch28-29/RConn3 -- Branch26-29/RConn3
  Transformer9-29/RConn1 -- Branch9-29/LConn1
  Transformer9-29/RConn2 -- Branch9-29/LConn2
  Transformer9-29/RConn3 -- Branch9-29/LConn3
  Bus9/RConn1 -- Transformer9-29/LConn1
  Bus9/RConn2 -- Transformer9-29/LConn2
  Bus9/RConn3 -- Transformer9-29/LConn3
  Branch10-31/RConn1 -- Bus31/RConn1 -- Branch31-31/LConn1 -- Branch31-53/LConn1 -- Branch31-38/LConn1 -- Branch30-31/RConn1
  Branch10-31/RConn2 -- Bus31/RConn2 -- Branch31-31/LConn2 -- Branch31-53/LConn2 -- Branch31-38/LConn2 -- Branch30-31/RConn2
  Branch10-31/RConn3 -- Bus31/RConn3 -- Branch31-31/LConn3 -- Branch31-53/LConn3 -- Branch31-38/LConn3 -- Branch30-31/RConn3
  Transformer10-31/RConn1 -- Branch10-31/LConn1
  Transformer10-31/RConn2 -- Branch10-31/LConn2
  Transformer10-31/RConn3 -- Branch10-31/LConn3
  Bus10/RConn1 -- Transformer10-31/LConn1
  Bus10/RConn2 -- Transformer10-31/LConn2
  Bus10/RConn3 -- Transformer10-31/LConn3
  Branch11-32/RConn1 -- Bus32/RConn1 -- Branch32-32/LConn1 -- Branch32-33/LConn1 -- Branch30-32/RConn1
  Branch11-32/RConn2 -- Bus32/RConn2 -- Branch32-32/LConn2 -- Branch32-33/LConn2 -- Branch30-32/RConn2
  Branch11-32/RConn3 -- Bus32/RConn3 -- Branch32-32/LConn3 -- Branch32-33/LConn3 -- Branch30-32/RConn3
  Transformer11-32/RConn1 -- Branch11-32/LConn1
  Transformer11-32/RConn2 -- Branch11-32/LConn2
  Transformer11-32/RConn3 -- Branch11-32/LConn3
  Bus11/RConn1 -- Transformer11-32/LConn1
  Bus11/RConn2 -- Transformer11-32/LConn2
  Bus11/RConn3 -- Transformer11-32/LConn3
  Branch12-36/RConn1 -- Bus36/RConn1 -- Branch36-36/LConn1 -- Branch36-61/LConn1 -- Branch34-36/RConn1 -- Branch17-36/RConn1
  Branch12-36/RConn2 -- Bus36/RConn2 -- Branch36-36/LConn2 -- Branch36-61/LConn2 -- Branch34-36/RConn2 -- Branch17-36/RConn2
  Branch12-36/RConn3 -- Bus36/RConn3 -- Branch36-36/LConn3 -- Branch36-61/LConn3 -- Branch34-36/RConn3 -- Branch17-36/RConn3
  Transformer12-36/RConn1 -- Branch12-36/LConn1
  Transformer12-36/RConn2 -- Branch12-36/LConn2
  Transformer12-36/RConn3 -- Branch12-36/LConn3
  Bus12/RConn1 -- Transformer12-36/LConn1
  Bus12/RConn2 -- Transformer12-36/LConn2
  Bus12/RConn3 -- Transformer12-36/LConn3
  Branch13-17/RConn1 -- Bus17/RConn1 -- Branch17-17/LConn1 -- Branch17-43/LConn1 -- Branch17-36/LConn1
  Branch13-17/RConn2 -- Bus17/RConn2 -- Branch17-17/LConn2 -- Branch17-43/LConn2 -- Branch17-36/LConn2
  Branch13-17/RConn3 -- Bus17/RConn3 -- Branch17-17/LConn3 -- Branch17-43/LConn3 -- Branch17-36/LConn3
  Transformer13-17/RConn1 -- Branch13-17/LConn1
  Transformer13-17/RConn2 -- Branch13-17/LConn2
  Transformer13-17/RConn3 -- Branch13-17/LConn3
  Bus13/RConn1 -- Transformer13-17/LConn1
  Bus13/RConn2 -- Transformer13-17/LConn2
  Bus13/RConn3 -- Transformer13-17/LConn3
  Branch14-41/RConn1 -- Bus41/RConn1 -- Branch41-41/LConn1 -- Branch41-42/LConn1 -- Branch40-41/RConn1
  Branch14-41/RConn2 -- Bus41/RConn2 -- Branch41-41/LConn2 -- Branch41-42/LConn2 -- Branch40-41/RConn2
  Branch14-41/RConn3 -- Bus41/RConn3 -- Branch41-41/LConn3 -- Branch41-42/LConn3 -- Branch40-41/RConn3
  Bus14/RConn1 -- Branch14-41/LConn1
  Bus14/RConn2 -- Branch14-41/LConn2
  Bus14/RConn3 -- Branch14-41/LConn3
  Branch15-42/RConn1 -- Bus42/RConn1 -- Branch42-42/LConn1 -- Branch41-42/RConn1 -- Branch18-42/RConn1
  Branch15-42/RConn2 -- Bus42/RConn2 -- Branch42-42/LConn2 -- Branch41-42/RConn2 -- Branch18-42/RConn2
  Branch15-42/RConn3 -- Bus42/RConn3 -- Branch42-42/LConn3 -- Branch41-42/RConn3 -- Branch18-42/RConn3
  Bus15/RConn1 -- Branch15-42/LConn1
  Bus15/RConn2 -- Branch15-42/LConn2
  Bus15/RConn3 -- Branch15-42/LConn3
  Branch16-54/RConn1 -- Bus54/RConn1 -- Branch54-54/LConn1 -- Branch54-55/LConn1 -- Branch53-54/RConn1 -- Branch25-54/RConn1
  Branch16-54/RConn2 -- Bus54/RConn2 -- Branch54-54/LConn2 -- Branch54-55/LConn2 -- Branch53-54/RConn2 -- Branch25-54/RConn2
  Branch16-54/RConn3 -- Bus54/RConn3 -- Branch54-54/LConn3 -- Branch54-55/LConn3 -- Branch53-54/RConn3 -- Branch25-54/RConn3
  Transformer16-54/RConn1 -- Branch16-54/LConn1
  Transformer16-54/RConn2 -- Branch16-54/LConn2
  Transformer16-54/RConn3 -- Branch16-54/LConn3
  Bus16/RConn1 -- Transformer16-54/LConn1
  Bus16/RConn2 -- Transformer16-54/LConn2
  Bus16/RConn3 -- Transformer16-54/LConn3
  Branch17-43/RConn1 -- Bus43/RConn1 -- Branch43-44/LConn1
  Branch17-43/RConn2 -- Bus43/RConn2 -- Branch43-44/LConn2
  Branch17-43/RConn3 -- Bus43/RConn3 -- Branch43-44/LConn3
  Branch18-49/RConn1 -- Bus49/RConn1 -- Branch49-49/LConn1 -- Branch46-49/RConn1
  Branch18-49/RConn2 -- Bus49/RConn2 -- Branch49-49/LConn2 -- Branch46-49/RConn2
  Branch18-49/RConn3 -- Bus49/RConn3 -- Branch49-49/LConn3 -- Branch46-49/RConn3
  Branch18-50/RConn1 -- Bus50/RConn1 -- Branch50-50/LConn1 -- Branch50-51/LConn1
  Branch18-50/RConn2 -- Bus50/RConn2 -- Branch50-50/LConn2 -- Branch50-51/LConn2
  Branch18-50/RConn3 -- Bus50/RConn3 -- Branch50-50/LConn3 -- Branch50-51/LConn3
  Transformer19-20/RConn1 -- Branch19-20/LConn1
  Transformer19-20/RConn2 -- Branch19-20/LConn2
  Transformer19-20/RConn3 -- Branch19-20/LConn3
  Branch19-68/RConn1 -- Bus68/RConn1 -- Branch68-68/LConn1 -- Branch67-68/RConn1 -- Branch37-68/RConn1 -- Branch24-68/RConn1 -- Branch21-68/RConn1
  Branch19-68/RConn2 -- Bus68/RConn2 -- Branch68-68/LConn2 -- Branch67-68/RConn2 -- Branch37-68/RConn2 -- Branch24-68/RConn2 -- Branch21-68/RConn2
  Branch19-68/RConn3 -- Bus68/RConn3 -- Branch68-68/LConn3 -- Branch67-68/RConn3 -- Branch37-68/RConn3 -- Branch24-68/RConn3 -- Branch21-68/RConn3
  Branch21-22/LConn1 -- Bus21/RConn1 -- Branch21-21/LConn1 -- Branch21-68/LConn1
  Branch21-22/LConn2 -- Bus21/RConn2 -- Branch21-21/LConn2 -- Branch21-68/LConn2
  Branch21-22/LConn3 -- Bus21/RConn3 -- Branch21-21/LConn3 -- Branch21-68/LConn3
  Branch23-24/RConn1 -- Bus24/RConn1 -- Branch24-24/LConn1 -- Branch24-68/LConn1
  Branch23-24/RConn2 -- Bus24/RConn2 -- Branch24-24/LConn2 -- Branch24-68/LConn2
  Branch23-24/RConn3 -- Bus24/RConn3 -- Branch24-24/LConn3 -- Branch24-68/LConn3
  Branch25-26/RConn1 -- Bus26/RConn1 -- Branch26-26/LConn1 -- Branch26-29/LConn1 -- Branch26-28/LConn1 -- Branch26-27/LConn1
  Branch25-26/RConn2 -- Bus26/RConn2 -- Branch26-26/LConn2 -- Branch26-29/LConn2 -- Branch26-28/LConn2 -- Branch26-27/LConn2
  Branch25-26/RConn3 -- Bus26/RConn3 -- Branch26-26/LConn3 -- Branch26-29/LConn3 -- Branch26-28/LConn3 -- Branch26-27/LConn3
  Branch26-27/RConn1 -- Bus27/RConn1 -- Branch27-27/LConn1 -- Branch27-53/LConn1 -- Branch27-37/LConn1
  Branch26-27/RConn2 -- Bus27/RConn2 -- Branch27-27/LConn2 -- Branch27-53/LConn2 -- Branch27-37/LConn2
  Branch26-27/RConn3 -- Bus27/RConn3 -- Branch27-27/LConn3 -- Branch27-53/LConn3 -- Branch27-37/LConn3
  Branch26-28/RConn1 -- Bus28/RConn1 -- Branch28-28/LConn1 -- Branch28-29/LConn1
  Branch26-28/RConn2 -- Bus28/RConn2 -- Branch28-28/LConn2 -- Branch28-29/LConn2
  Branch26-28/RConn3 -- Bus28/RConn3 -- Branch28-28/LConn3 -- Branch28-29/LConn3
  Branch27-37/RConn1 -- Bus37/RConn1 -- Branch37-37/LConn1 -- Branch37-68/LConn1 -- Branch37-52/LConn1
  Branch27-37/RConn2 -- Bus37/RConn2 -- Branch37-37/LConn2 -- Branch37-68/LConn2 -- Branch37-52/LConn2
  Branch27-37/RConn3 -- Bus37/RConn3 -- Branch37-37/LConn3 -- Branch37-68/LConn3 -- Branch37-52/LConn3
  Branch27-53/RConn1 -- Bus53/RConn1 -- Branch53-53/LConn1 -- Branch53-54/LConn1 -- Branch47-53/RConn1 -- Branch31-53/RConn1 -- Branch30-53/RConn1
  Branch27-53/RConn2 -- Bus53/RConn2 -- Branch53-53/LConn2 -- Branch53-54/LConn2 -- Branch47-53/RConn2 -- Branch31-53/RConn2 -- Branch30-53/RConn2
  Branch27-53/RConn3 -- Bus53/RConn3 -- Branch53-53/LConn3 -- Branch53-54/LConn3 -- Branch47-53/RConn3 -- Branch31-53/RConn3 -- Branch30-53/RConn3
  Branch30-31/LConn1 -- Bus30/RConn1 -- Branch30-30/LConn1 -- Branch30-61/LConn1 -- Branch30-53/LConn1 -- Branch30-32/LConn1
  Branch30-31/LConn2 -- Bus30/RConn2 -- Branch30-30/LConn2 -- Branch30-61/LConn2 -- Branch30-53/LConn2 -- Branch30-32/LConn2
  Branch30-31/LConn3 -- Bus30/RConn3 -- Branch30-30/LConn3 -- Branch30-61/LConn3 -- Branch30-53/LConn3 -- Branch30-32/LConn3
  Branch30-61/RConn1 -- Bus61/RConn1 -- Branch61-61/LConn1 -- Branch60-61/RConn1 -- Branch36-61/RConn1
  Branch30-61/RConn2 -- Bus61/RConn2 -- Branch61-61/LConn2 -- Branch60-61/RConn2 -- Branch36-61/RConn2
  Branch30-61/RConn3 -- Bus61/RConn3 -- Branch61-61/LConn3 -- Branch60-61/RConn3 -- Branch36-61/RConn3
  Branch31-38/RConn1 -- Bus38/RConn1 -- Branch38-38/LConn1 -- Branch38-46/LConn1 -- Branch33-38/RConn1
  Branch31-38/RConn2 -- Bus38/RConn2 -- Branch38-38/LConn2 -- Branch38-46/LConn2 -- Branch33-38/RConn2
  Branch31-38/RConn3 -- Bus38/RConn3 -- Branch38-38/LConn3 -- Branch38-46/LConn3 -- Branch33-38/RConn3
  Branch32-33/RConn1 -- Bus33/RConn1 -- Branch33-33/LConn1 -- Branch33-38/LConn1 -- Branch33-34/LConn1
  Branch32-33/RConn2 -- Bus33/RConn2 -- Branch33-33/LConn2 -- Branch33-38/LConn2 -- Branch33-34/LConn2
  Branch32-33/RConn3 -- Bus33/RConn3 -- Branch33-33/LConn3 -- Branch33-38/LConn3 -- Branch33-34/LConn3
  Branch33-34/RConn1 -- Bus34/RConn1 -- Branch34-34/LConn1 -- Branch34-36/LConn1 -- Transformer34-35/LConn1
  Branch33-34/RConn2 -- Bus34/RConn2 -- Branch34-34/LConn2 -- Branch34-36/LConn2 -- Transformer34-35/LConn2
  Branch33-34/RConn3 -- Bus34/RConn3 -- Branch34-34/LConn3 -- Branch34-36/LConn3 -- Transformer34-35/LConn3
  Branch34-35/RConn1 -- Bus35/RConn1 -- Branch35-35/LConn1 -- Branch35-45/LConn1
  Branch34-35/RConn2 -- Bus35/RConn2 -- Branch35-35/LConn2 -- Branch35-45/LConn2
  Branch34-35/RConn3 -- Bus35/RConn3 -- Branch35-35/LConn3 -- Branch35-45/LConn3
  Transformer34-35/RConn1 -- Branch34-35/LConn1
  Transformer34-35/RConn2 -- Branch34-35/LConn2
  Transformer34-35/RConn3 -- Branch34-35/LConn3
  Branch35-45/RConn1 -- Bus45/RConn1 -- Branch45-45/LConn1 -- Branch45-51/LConn1 -- Branch44-45/RConn1 -- Branch39-45/RConn1
  Branch35-45/RConn2 -- Bus45/RConn2 -- Branch45-45/LConn2 -- Branch45-51/LConn2 -- Branch44-45/RConn2 -- Branch39-45/RConn2
  Branch35-45/RConn3 -- Bus45/RConn3 -- Branch45-45/LConn3 -- Branch45-51/LConn3 -- Branch44-45/RConn3 -- Branch39-45/RConn3
  Branch37-52/RConn1 -- Bus52/RConn1 -- Branch52-52/LConn1 -- Branch52-55/LConn1
  Branch37-52/RConn2 -- Bus52/RConn2 -- Branch52-52/LConn2 -- Branch52-55/LConn2
  Branch37-52/RConn3 -- Bus52/RConn3 -- Branch52-52/LConn3 -- Branch52-55/LConn3
  Branch38-46/RConn1 -- Bus46/RConn1 -- Branch46-46/LConn1 -- Branch46-49/LConn1
  Branch38-46/RConn2 -- Bus46/RConn2 -- Branch46-46/LConn2 -- Branch46-49/LConn2
  Branch38-46/RConn3 -- Bus46/RConn3 -- Branch46-46/LConn3 -- Branch46-49/LConn3
  Branch39-44/RConn1 -- Bus44/RConn1 -- Branch44-44/LConn1 -- Branch44-45/LConn1 -- Branch43-44/RConn1
  Branch39-44/RConn2 -- Bus44/RConn2 -- Branch44-44/LConn2 -- Branch44-45/LConn2 -- Branch43-44/RConn2
  Branch39-44/RConn3 -- Bus44/RConn3 -- Branch44-44/LConn3 -- Branch44-45/LConn3 -- Branch43-44/RConn3
  Branch39-44/LConn1 -- Bus39/RConn1 -- Branch39-39/LConn1 -- Branch39-45/LConn1
  Branch39-44/LConn2 -- Bus39/RConn2 -- Branch39-39/LConn2 -- Branch39-45/LConn2
  Branch39-44/LConn3 -- Bus39/RConn3 -- Branch39-39/LConn3 -- Branch39-45/LConn3
  Branch40-41/LConn1 -- Bus40/RConn1 -- Branch40-40/LConn1 -- Branch40-48/LConn1
  Branch40-41/LConn2 -- Bus40/RConn2 -- Branch40-40/LConn2 -- Branch40-48/LConn2
  Branch40-41/LConn3 -- Bus40/RConn3 -- Branch40-40/LConn3 -- Branch40-48/LConn3
  Branch40-48/RConn1 -- Bus48/RConn1 -- Branch48-48/LConn1 -- Branch47-48/RConn1
  Branch40-48/RConn2 -- Bus48/RConn2 -- Branch48-48/LConn2 -- Branch47-48/RConn2
  Branch40-48/RConn3 -- Bus48/RConn3 -- Branch48-48/LConn3 -- Branch47-48/RConn3
  Branch45-51/RConn1 -- Bus51/RConn1 -- Branch51-51/LConn1 -- Branch50-51/RConn1
  Branch45-51/RConn2 -- Bus51/RConn2 -- Branch51-51/LConn2 -- Branch50-51/RConn2
  Branch45-51/RConn3 -- Bus51/RConn3 -- Branch51-51/LConn3 -- Branch50-51/RConn3
  Branch47-48/LConn1 -- Bus47/RConn1 -- Branch47-47/LConn1 -- Branch47-53/LConn1
  Branch47-48/LConn2 -- Bus47/RConn2 -- Branch47-47/LConn2 -- Branch47-53/LConn2
  Branch47-48/LConn3 -- Bus47/RConn3 -- Branch47-47/LConn3 -- Branch47-53/LConn3
  Branch52-55/RConn1 -- Bus55/RConn1 -- Branch55-55/LConn1 -- Branch55-56/LConn1 -- Branch54-55/RConn1
  Branch52-55/RConn2 -- Bus55/RConn2 -- Branch55-55/LConn2 -- Branch55-56/LConn2 -- Branch54-55/RConn2
  Branch52-55/RConn3 -- Bus55/RConn3 -- Branch55-55/LConn3 -- Branch55-56/LConn3 -- Branch54-55/RConn3
  Branch55-56/RConn1 -- Bus56/RConn1 -- Branch56-56/LConn1 -- Branch56-66/LConn1 -- Branch56-57/LConn1
  Branch55-56/RConn2 -- Bus56/RConn2 -- Branch56-56/LConn2 -- Branch56-66/LConn2 -- Branch56-57/LConn2
  Branch55-56/RConn3 -- Bus56/RConn3 -- Branch56-56/LConn3 -- Branch56-66/LConn3 -- Branch56-57/LConn3
  Branch56-57/RConn1 -- Bus57/RConn1 -- Branch57-57/LConn1 -- Branch57-60/LConn1 -- Branch57-58/LConn1
  Branch56-57/RConn2 -- Bus57/RConn2 -- Branch57-57/LConn2 -- Branch57-60/LConn2 -- Branch57-58/LConn2
  Branch56-57/RConn3 -- Bus57/RConn3 -- Branch57-57/LConn3 -- Branch57-60/LConn3 -- Branch57-58/LConn3
  Branch56-66/RConn1 -- Bus66/RConn1 -- Branch66-66/LConn1 -- Branch66-67/LConn1 -- Branch65-66/RConn1
  Branch56-66/RConn2 -- Bus66/RConn2 -- Branch66-66/LConn2 -- Branch66-67/LConn2 -- Branch65-66/RConn2
  Branch56-66/RConn3 -- Bus66/RConn3 -- Branch66-66/LConn3 -- Branch66-67/LConn3 -- Branch65-66/RConn3
  Branch57-60/RConn1 -- Bus60/RConn1 -- Branch60-60/LConn1 -- Branch60-61/LConn1 -- Branch59-60/RConn1
  Branch57-60/RConn2 -- Bus60/RConn2 -- Branch60-60/LConn2 -- Branch60-61/LConn2 -- Branch59-60/RConn2
  Branch57-60/RConn3 -- Bus60/RConn3 -- Branch60-60/LConn3 -- Branch60-61/LConn3 -- Branch59-60/RConn3
  Branch58-59/RConn1 -- Bus59/RConn1 -- Branch59-59/LConn1 -- Branch59-60/LConn1
  Branch58-59/RConn2 -- Bus59/RConn2 -- Branch59-59/LConn2 -- Branch59-60/LConn2
  Branch58-59/RConn3 -- Bus59/RConn3 -- Branch59-59/LConn3 -- Branch59-60/LConn3
  Branch58-63/RConn1 -- Bus63/RConn1 -- Branch63-63/LConn1 -- Transformer63-64/LConn1 -- Branch62-63/RConn1
  Branch58-63/RConn2 -- Bus63/RConn2 -- Branch63-63/LConn2 -- Transformer63-64/LConn2 -- Branch62-63/RConn2
  Branch58-63/RConn3 -- Bus63/RConn3 -- Branch63-63/LConn3 -- Transformer63-64/LConn3 -- Branch62-63/RConn3
  Branch62-65/RConn1 -- Bus65/RConn1 -- Branch65-65/LConn1 -- Branch65-66/LConn1 -- Branch64-65/RConn1
  Branch62-65/RConn2 -- Bus65/RConn2 -- Branch65-65/LConn2 -- Branch65-66/LConn2 -- Branch64-65/RConn2
  Branch62-65/RConn3 -- Bus65/RConn3 -- Branch65-65/LConn3 -- Branch65-66/LConn3 -- Branch64-65/RConn3
  Branch63-64/RConn1 -- Bus64/RConn1 -- Branch64-64/LConn1 -- Transformer64-65/LConn1
  Branch63-64/RConn2 -- Bus64/RConn2 -- Branch64-64/LConn2 -- Transformer64-65/LConn2
  Branch63-64/RConn3 -- Bus64/RConn3 -- Branch64-64/LConn3 -- Transformer64-65/LConn3
  Transformer63-64/RConn1 -- Branch63-64/LConn1
  Transformer63-64/RConn2 -- Branch63-64/LConn2
  Transformer63-64/RConn3 -- Branch63-64/LConn3
  Transformer64-65/RConn1 -- Branch64-65/LConn1
  Transformer64-65/RConn2 -- Branch64-65/LConn2
  Transformer64-65/RConn3 -- Branch64-65/LConn3
  Branch66-67/RConn1 -- Bus67/RConn1 -- Branch67-67/LConn1 -- Branch67-68/LConn1
  Branch66-67/RConn2 -- Bus67/RConn2 -- Branch67-67/LConn2 -- Branch67-68/LConn2
  Branch66-67/RConn3 -- Bus67/RConn3 -- Branch67-67/LConn3 -- Branch67-68/LConn3
  SM1/LConn1 -- Bus1/LConn1
  SM1/LConn2 -- Bus1/LConn2
  SM1/LConn3 -- Bus1/LConn3
  SM2/LConn1 -- Bus2/LConn1
  SM2/LConn2 -- Bus2/LConn2
  SM2/LConn3 -- Bus2/LConn3
  SM3/LConn1 -- Bus3/LConn1
  SM3/LConn2 -- Bus3/LConn2
  SM3/LConn3 -- Bus3/LConn3
  SM4/LConn1 -- Bus4/LConn1
  SM4/LConn2 -- Bus4/LConn2
  SM4/LConn3 -- Bus4/LConn3
  SM5/LConn1 -- Bus5/LConn1
  SM5/LConn2 -- Bus5/LConn2
  SM5/LConn3 -- Bus5/LConn3
  SM6/LConn1 -- Bus6/LConn1
  SM6/LConn2 -- Bus6/LConn2
  SM6/LConn3 -- Bus6/LConn3
  SM7/LConn1 -- Bus7/LConn1
  SM7/LConn2 -- Bus7/LConn2
  SM7/LConn3 -- Bus7/LConn3
  SM8/LConn1 -- Bus8/LConn1
  SM8/LConn2 -- Bus8/LConn2
  SM8/LConn3 -- Bus8/LConn3
  SM9/LConn1 -- Bus9/LConn1
  SM9/LConn2 -- Bus9/LConn2
  SM9/LConn3 -- Bus9/LConn3
  SM10/LConn1 -- Bus10/LConn1
  SM10/LConn2 -- Bus10/LConn2
  SM10/LConn3 -- Bus10/LConn3
  SM11/LConn1 -- Bus11/LConn1
  SM11/LConn2 -- Bus11/LConn2
  SM11/LConn3 -- Bus11/LConn3
  SM12/LConn1 -- Bus12/LConn1
  SM12/LConn2 -- Bus12/LConn2
  SM12/LConn3 -- Bus12/LConn3
  SM13/LConn1 -- Bus13/LConn1
  SM13/LConn2 -- Bus13/LConn2
  SM13/LConn3 -- Bus13/LConn3
  SM14/LConn1 -- Bus14/LConn1
  SM14/LConn2 -- Bus14/LConn2
  SM14/LConn3 -- Bus14/LConn3
  SM15/LConn1 -- Bus15/LConn1
  SM15/LConn2 -- Bus15/LConn2
  SM15/LConn3 -- Bus15/LConn3
  SM16/LConn1 -- Bus16/LConn1
  SM16/LConn2 -- Bus16/LConn2
  SM16/LConn3 -- Bus16/LConn3
  Load Impulse1/LConn3 -- Current Measurement1/RConn1
  D-GND22/LConn1 -- Load Impulse1/RConn1
  Bus37/LConn2 -- Load Impulse1/LConn2
  Bus37/LConn1 -- Load Impulse1/LConn1
  Bus37/LConn3 -- Current Measurement1/LConn1
